simulink model "v2012_PF"  (Simulink 7.6)
(part 1 of 4)
settings: Solver=ode45  StartTime=0.0  StopTime=10.0  RelTol=1e-3
libraries: fm_lib x1
settings Model: Creator=davidusb  LastModifiedBy=davidusb

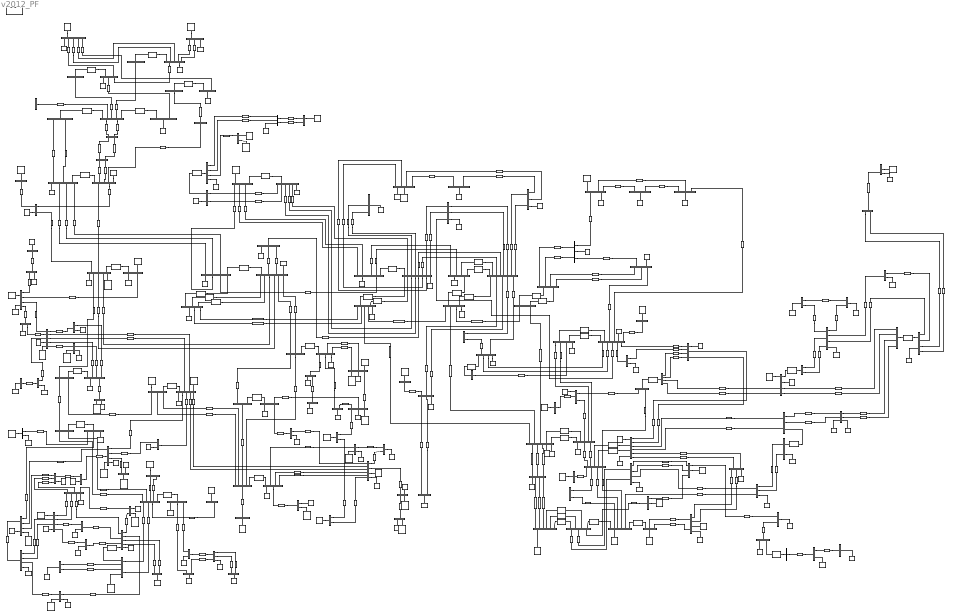
== system v2012_PF ==
  note: Hacia Empresas
      | Mixtas PDVSA
  note: REACTOR
      | 3x300
  note: REACTOR
      | 4x300
  note: COMP
      | ESTATICO
  note: REACTOR
      | 2x50
  note: Guri 400 kV
  note: Macagua I y III
  note: Caruachi
  note: Macagua II
  note: S/E San Geronimo 765kV
  note: S/E Malena 765kV
  note: S/E Guri 765kV
  note: Ciudad
      | Guayana
  note: Guri 230 kV
  note: (AT adicional 150MVA 2012)
  note: 2x100MVAr
      | SHUNT CAP
  note: Puerto La Cruz
  note: Caracas
  note: Maracay
  note: S/E Sur 765kV
  note: REACTOR
      | 2x100
  note: (2da linea 2012)
  note: Valencia
  note: S/E La Horqueta 765kV
  note: S/E La Arenosa 765kV
  note: LIBRE
  note: Elaborado por: Ing. David Hernández Torres, PhD
      |
      | VERSION: 29 de Noviembre de 2012 (Simplificada, niveles de tensión: 765, 400 y 230 kV)
      | (Solo se consideran una pequeña parte de la red oriental y la red de Los Andes en 115kV)
      |
      | Fuentes:
      | Elaborado siguiendo diagrama unifilar actualizado hasta el 2003 (OPSIS) y las actualizaciones
      | del sistema descritas en el Anuario Estadístico del MPPEE hasta el año 2010 y en los
      | informe anuales OPSIS 2005-2008. Finalmente el modelo 2012 se obtiene luego de actualización
      | del modelo 2010 bajo las premisas descritas en los archivos pronostico_demanda_electrica.xls y
      | Datos SEN.xls
      |
      | (Es necesaria la instalación del toolbox PSAT, el esquema se elaboró con Simulink
      | y la version 7.11 R2010b de Matlab, se puede ejecutar el archivo de datos .m desde Octave y la
      | version de PSAT correspondiente)
  note: SISTEMA ELECTRICO NACIONAL
  note: COMP
      | ESTATICO
  note: REACTOR
      | 2x50
  note: REACTOR
      | 1x300
  note: REACTOR
      | 2x25
  note: Cumana
  note: REACTOR
      | 1x50
  note: Isla de Margarita
  note: REACTOR
      | 2x25
  note: Brasil
  note: REACTOR
      | 2x50
  note: TAP=1.1
  note: Termozulia
      | Rafael Urdaneta
  note: CAPACITOR
      | 1x108
  note: REACTOR
      | 1x50
  note: REACTOR
      | 4x50
  note: SERIES
      | CAPACITOR
      | COMP
      | 3x50 OHM
  note: Maracaibo
  note: HACIA COLOMBIA
  note: REACTOR
      | 1x300
  note: REACTOR
      | 4x50
  note: LIBRE
  note: LIBRE
  note: S/E Yaracuy 765kV
  note: Barquisimeto
  note: Merida
  note: San Cristobal
  note: Colombia
  note: REACTOR
      | 2x20
  note: Peninsula de Paraguaná
  note: (2da linea 2012)
  note: (Entrada de 257MW en 2013)
      | Fabricio Ojeda
  note: Equivalente
      | hacia Cabudare
  note: Equivalente
      | hacia Cabimas -
      | El Tablazo
  Acarigua I : PMComponent  Tag=PSATblock  Description=Connection  PhysicalDomain=psatdomain  LeftPortType=p1  RightPortType=p1  LConnTagsString=__newl0|__newl1|__newl2  RConnTagsString=__newr0|__newr1|__newr2  mask(Bus){in=3, out=3, p2q=115, p3_4q=[0.98444    -0.26004], p5q=1, p6q=1}
      mask prompts: in "Number of inputs:"; out "Number of outputs:"; p2q "Voltage Rating [kV]"; p3_4q "Voltage initial guess [p.u.  rad]"; p5q "Area number"; p6q "Region number"
      mask help: Bus block.
      mask init:
      | fm_inout
      settings: AttributesFormatString="|V| =  0.9513 p.u.\\n<V  = -0.0895 rad"
      mask CallbackString: ||||fm_block|
      mask Display: plot([0 1 1 0 0],[0 0 1 1 0])
  Acarigua II 115kV : PMComponent  Tag=PSATblock  Description=Connection  PhysicalDomain=psatdomain  LeftPortType=p1  RightPortType=p1  LConnTagsString=__newl0|__newl1|__newl2  RConnTagsString=__newr0|__newr1|__newr2|__newr3  mask(Bus){in=3, out=4, p2q=115, p3_4q=[0.98444    -0.26004], p5q=1, p6q=1}
      mask prompts: in "Number of inputs:"; out "Number of outputs:"; p2q "Voltage Rating [kV]"; p3_4q "Voltage initial guess [p.u.  rad]"; p5q "Area number"; p6q "Region number"
      mask help: Bus block.
      mask init:
      | fm_inout
      settings: AttributesFormatString="|V| =  0.9304 p.u.\\n<V  = -0.1031 rad"
      mask CallbackString: ||||fm_block|
      mask Display: plot([0 1 1 0 0],[0 0 1 1 0])
  Acarigua II 230kV : PMComponent  Tag=PSATblock  Description=Connection  PhysicalDomain=psatdomain  LeftPortType=p1  RightPortType=p1  LConnTagsString=__newl0|__newl1|__newl2  RConnTagsString=__newr0|__newr1|__newr2  mask(Bus){in=3, out=3, p2q=230, p3_4q=[0.96856    -0.61292], p5q=1, p6q=1}
      mask prompts: in "Number of inputs:"; out "Number of outputs:"; p2q "Voltage Rating [kV]"; p3_4q "Voltage initial guess [p.u.  rad]"; p5q "Area number"; p6q "Region number"
      mask help: Bus block.
      mask init:
      | fm_inout
      settings: AttributesFormatString="|V| =  0.9644 p.u.\\n<V  = -0.0672 rad"
      mask CallbackString: ||||fm_block|
      mask Display: plot([0 1 1 0 0],[0 0 1 1 0])
  Aragua 230kV : PMComponent  Tag=PSATblock  Description=Connection  PhysicalDomain=psatdomain  LeftPortType=p1  RightPortType=p1  LConnTagsString=__newl0|__newl1|__newl2  RConnTagsString=__newr0|__newr1|__newr2  mask(Bus){in=3, out=3, p2q=230, p3_4q=[0.953    -0.54917], p5q=1, p6q=1}
      mask prompts: in "Number of inputs:"; out "Number of outputs:"; p2q "Voltage Rating [kV]"; p3_4q "Voltage initial guess [p.u.  rad]"; p5q "Area number"; p6q "Region number"
      mask help: Bus block.
      mask init:
      | fm_inout
      settings: AttributesFormatString="|V| =  0.9696 p.u.\\n<V  = -0.2355 rad"
      mask CallbackString: ||||fm_block|
      mask Display: plot([0 1 1 0 0],[0 0 1 1 0])
  Araure : PMComponent  Tag=PSATblock  Description=Connection  PhysicalDomain=psatdomain  LeftPortType=p1  RightPortType=p1  LConnTagsString=__newl0|__newl1  RConnTagsString=__newr0  mask(Bus){in=2, out=1, p2q=115, p3_4q=[1.0023    -0.25717], p5q=1, p6q=1}
      mask prompts: in "Number of inputs:"; out "Number of outputs:"; p2q "Voltage Rating [kV]"; p3_4q "Voltage initial guess [p.u.  rad]"; p5q "Area number"; p6q "Region number"
      mask help: Bus block.
      mask init:
      | fm_inout
      settings: AttributesFormatString="|V| =  0.9284 p.u.\\n<V  = -0.0990 rad"
      mask CallbackString: ||||fm_block|
      mask Display: plot([0 1 1 0 0],[0 0 1 1 0])
  Auto1 : PMComponent  Tag=PSATblock  Description=Power Flow  PhysicalDomain=psatdomain  LeftPortType=p1  RightPortType=p1  LConnTagsString=__newl0  RConnTagsString=__newr0  mask(Line){p3_4_5q=[1500  765 60], p7q=1.9124, p8q=0.003, p9q=0.148, p13_14_15q=[0.0  0.0  0.0], p16q=on}
      mask prompts: p3_4_5q "Power, Voltage and Frequency Ratings [MVA, kV, Hz]"; p7q "Primary and secondary voltage ratio [kV/kV]"; p8q "Resistance [p.u.]"; p9q "Reactance [p.u.]"; p13_14_15q "Imax, Pmax and Smax [p.u., p.u., p.u.]"; p16q "Connected"
      mask help: This block defines an auto-transformer.
      mask init:
      | [x,y] = fm_draw('circle');
      | [xq,yq] = fm_draw('quarter');
      mask CallbackString: |||||fm_block
      mask Display: plot(x,y,1.75*xq,yq,[-1 -1.3],[0 0],[1.75 2.05],[0 0])
  Auto10 : PMComponent  Tag=PSATblock  Description=Power Flow  PhysicalDomain=psatdomain  LeftPortType=p1  RightPortType=p1  LConnTagsString=__newl0  RConnTagsString=__newr0  mask(Line){p3_4_5q=[200  230 60], p7q=2, p8q=0.01, p9q=0.16, p13_14_15q=[0.0  0.0  0.0], p16q=on}
      mask prompts: p3_4_5q "Power, Voltage and Frequency Ratings [MVA, kV, Hz]"; p7q "Primary and secondary voltage ratio [kV/kV]"; p8q "Resistance [p.u.]"; p9q "Reactance [p.u.]"; p13_14_15q "Imax, Pmax and Smax [p.u., p.u., p.u.]"; p16q "Connected"
      mask help: This block defines an auto-transformer.
      mask init:
      | [x,y] = fm_draw('circle');
      | [xq,yq] = fm_draw('quarter');
      mask CallbackString: |||||fm_block
      mask Display: plot(x,y,1.75*xq,yq,[-1 -1.3],[0 0],[1.75 2.05],[0 0])
  Auto11 : PMComponent  Tag=PSATblock  Description=Power Flow  PhysicalDomain=psatdomain  LeftPortType=p1  RightPortType=p1  LConnTagsString=__newl0  RConnTagsString=__newr0  mask(Line){p3_4_5q=[900  400 60], p7q=1.7391, p8q=0.0024, p9q=0.10, p13_14_15q=[0.0  0.0  0.0], p16q=on}
      mask prompts: p3_4_5q "Power, Voltage and Frequency Ratings [MVA, kV, Hz]"; p7q "Primary and secondary voltage ratio [kV/kV]"; p8q "Resistance [p.u.]"; p9q "Reactance [p.u.]"; p13_14_15q "Imax, Pmax and Smax [p.u., p.u., p.u.]"; p16q "Connected"
      mask help: This block defines an auto-transformer.
      mask init:
      | [x,y] = fm_draw('circle');
      | [xq,yq] = fm_draw('quarter');
      mask CallbackString: |||||fm_block
      mask Display: plot(x,y,1.75*xq,yq,[-1 -1.3],[0 0],[1.75 2.05],[0 0])
  Auto12 : PMComponent  Tag=PSATblock  Description=Power Flow  PhysicalDomain=psatdomain  LeftPortType=p1  RightPortType=p1  LConnTagsString=__newl0  RConnTagsString=__newr0  mask(Line){p3_4_5q=[100  230 60], p7q=2, p8q=0.01, p9q=0.16, p13_14_15q=[0.0  0.0  0.0], p16q=on}
      mask prompts: p3_4_5q "Power, Voltage and Frequency Ratings [MVA, kV, Hz]"; p7q "Primary and secondary voltage ratio [kV/kV]"; p8q "Resistance [p.u.]"; p9q "Reactance [p.u.]"; p13_14_15q "Imax, Pmax and Smax [p.u., p.u., p.u.]"; p16q "Connected"
      mask help: This block defines an auto-transformer.
      mask init:
      | [x,y] = fm_draw('circle');
      | [xq,yq] = fm_draw('quarter');
      mask CallbackString: |||||fm_block
      mask Display: plot(x,y,1.75*xq,yq,[-1 -1.3],[0 0],[1.75 2.05],[0 0])
  Auto13 : PMComponent  Tag=PSATblock  Description=Power Flow  PhysicalDomain=psatdomain  LeftPortType=p1  RightPortType=p1  LConnTagsString=__newl0  RConnTagsString=__newr0  mask(Line){p3_4_5q=[200  230 60], p7q=2, p8q=0.01, p9q=0.16, p13_14_15q=[0.0  0.0  0.0], p16q=on}
      mask prompts: p3_4_5q "Power, Voltage and Frequency Ratings [MVA, kV, Hz]"; p7q "Primary and secondary voltage ratio [kV/kV]"; p8q "Resistance [p.u.]"; p9q "Reactance [p.u.]"; p13_14_15q "Imax, Pmax and Smax [p.u., p.u., p.u.]"; p16q "Connected"
      mask help: This block defines an auto-transformer.
      mask init:
      | [x,y] = fm_draw('circle');
      | [xq,yq] = fm_draw('quarter');
      mask CallbackString: |||||fm_block
      mask Display: plot(x,y,1.75*xq,yq,[-1 -1.3],[0 0],[1.75 2.05],[0 0])
  Auto14 : PMComponent  Tag=PSATblock  Description=Power Flow  PhysicalDomain=psatdomain  LeftPortType=p1  RightPortType=p1  LConnTagsString=__newl0  RConnTagsString=__newr0  mask(Line){p3_4_5q=[400  230 60], p7q=2, p8q=0.01, p9q=0.16, p13_14_15q=[0.0  0.0  0.0], p16q=on}
      mask prompts: p3_4_5q "Power, Voltage and Frequency Ratings [MVA, kV, Hz]"; p7q "Primary and secondary voltage ratio [kV/kV]"; p8q "Resistance [p.u.]"; p9q "Reactance [p.u.]"; p13_14_15q "Imax, Pmax and Smax [p.u., p.u., p.u.]"; p16q "Connected"
      mask help: This block defines an auto-transformer.
      mask init:
      | [x,y] = fm_draw('circle');
      | [xq,yq] = fm_draw('quarter');
      mask CallbackString: |||||fm_block
      mask Display: plot(x,y,1.75*xq,yq,[-1 -1.3],[0 0],[1.75 2.05],[0 0])
  Auto15 : PMComponent  Tag=PSATblock  Description=Power Flow  PhysicalDomain=psatdomain  LeftPortType=p1  RightPortType=p1  LConnTagsString=__newl0  RConnTagsString=__newr0  mask(Line){p3_4_5q=[1500  765 60], p7q=1.9124, p8q=0.003, p9q=0.148, p13_14_15q=[0.0  0.0  0.0], p16q=on}
      mask prompts: p3_4_5q "Power, Voltage and Frequency Ratings [MVA, kV, Hz]"; p7q "Primary and secondary voltage ratio [kV/kV]"; p8q "Resistance [p.u.]"; p9q "Reactance [p.u.]"; p13_14_15q "Imax, Pmax and Smax [p.u., p.u., p.u.]"; p16q "Connected"
      mask help: This block defines an auto-transformer.
      mask init:
      | [x,y] = fm_draw('circle');
      | [xq,yq] = fm_draw('quarter');
      mask CallbackString: |||||fm_block
      mask Display: plot(x,y,1.75*xq,yq,[-1 -1.3],[0 0],[1.75 2.05],[0 0])
  Auto16 : PMComponent  Tag=PSATblock  Description=Power Flow  PhysicalDomain=psatdomain  LeftPortType=p1  RightPortType=p1  LConnTagsString=__newl0  RConnTagsString=__newr0  mask(Line){p3_4_5q=[1000  400 60], p7q=1, p8q=0.001, p9q=0.0513, p13_14_15q=[0.0  0.0  0.0], p16q=on}
      mask prompts: p3_4_5q "Power, Voltage and Frequency Ratings [MVA, kV, Hz]"; p7q "Primary and secondary voltage ratio [kV/kV]"; p8q "Resistance [p.u.]"; p9q "Reactance [p.u.]"; p13_14_15q "Imax, Pmax and Smax [p.u., p.u., p.u.]"; p16q "Connected"
      mask help: This block defines an auto-transformer.
      mask init:
      | [x,y] = fm_draw('circle');
      | [xq,yq] = fm_draw('quarter');
      mask CallbackString: |||||fm_block
      mask Display: plot(x,y,1.75*xq,yq,[-1 -1.3],[0 0],[1.75 2.05],[0 0])
  Auto17 : PMComponent  Tag=PSATblock  Description=Power Flow  PhysicalDomain=psatdomain  LeftPortType=p1  RightPortType=p1  LConnTagsString=__newl0  RConnTagsString=__newr0  mask(Line){p3_4_5q=[450  400 60], p7q=1.7391, p8q=0.002, p9q=0.10, p13_14_15q=[0.0  0.0  0.0], p16q=on}
      mask prompts: p3_4_5q "Power, Voltage and Frequency Ratings [MVA, kV, Hz]"; p7q "Primary and secondary voltage ratio [kV/kV]"; p8q "Resistance [p.u.]"; p9q "Reactance [p.u.]"; p13_14_15q "Imax, Pmax and Smax [p.u., p.u., p.u.]"; p16q "Connected"
      mask help: This block defines an auto-transformer.
      mask init:
      | [x,y] = fm_draw('circle');
      | [xq,yq] = fm_draw('quarter');
      mask CallbackString: |||||fm_block
      mask Display: plot(x,y,1.75*xq,yq,[-1 -1.3],[0 0],[1.75 2.05],[0 0])
  Auto18 : PMComponent  Tag=PSATblock  Description=Power Flow  PhysicalDomain=psatdomain  LeftPortType=p1  RightPortType=p1  LConnTagsString=__newl0  RConnTagsString=__newr0  mask(Line){p3_4_5q=[450  400 60], p7q=1.7391, p8q=0.0011, p9q=0.0546, p13_14_15q=[0.0  0.0  0.0], p16q=on}
      mask prompts: p3_4_5q "Power, Voltage and Frequency Ratings [MVA, kV, Hz]"; p7q "Primary and secondary voltage ratio [kV/kV]"; p8q "Resistance [p.u.]"; p9q "Reactance [p.u.]"; p13_14_15q "Imax, Pmax and Smax [p.u., p.u., p.u.]"; p16q "Connected"
      mask help: This block defines an auto-transformer.
      mask init:
      | [x,y] = fm_draw('circle');
      | [xq,yq] = fm_draw('quarter');
      mask CallbackString: |||||fm_block
      mask Display: plot(x,y,1.75*xq,yq,[-1 -1.3],[0 0],[1.75 2.05],[0 0])
  Auto19 : PMComponent  Tag=PSATblock  Description=Power Flow  PhysicalDomain=psatdomain  LeftPortType=p1  RightPortType=p1  LConnTagsString=__newl0  RConnTagsString=__newr0  mask(Line){p3_4_5q=[1000  765 60], p7q=3.3256, p8q=0.003, p9q=0.15, p13_14_15q=[0.0  0.0  0.0], p16q=on}
      mask prompts: p3_4_5q "Power, Voltage and Frequency Ratings [MVA, kV, Hz]"; p7q "Primary and secondary voltage ratio [kV/kV]"; p8q "Resistance [p.u.]"; p9q "Reactance [p.u.]"; p13_14_15q "Imax, Pmax and Smax [p.u., p.u., p.u.]"; p16q "Connected"
      mask help: This block defines an auto-transformer.
      mask init:
      | [x,y] = fm_draw('circle');
      | [xq,yq] = fm_draw('quarter');
      mask CallbackString: |||||fm_block
      mask Display: plot(x,y,1.75*xq,yq,[-1 -1.3],[0 0],[1.75 2.05],[0 0])
  Auto2 : PMComponent  Tag=PSATblock  Description=Power Flow  PhysicalDomain=psatdomain  LeftPortType=p1  RightPortType=p1  LConnTagsString=__newl0  RConnTagsString=__newr0  mask(Line){p3_4_5q=[1500  765 60], p7q=1.9124, p8q=0.003, p9q=0.148, p13_14_15q=[0.0  0.0  0.0], p16q=on}
      mask prompts: p3_4_5q "Power, Voltage and Frequency Ratings [MVA, kV, Hz]"; p7q "Primary and secondary voltage ratio [kV/kV]"; p8q "Resistance [p.u.]"; p9q "Reactance [p.u.]"; p13_14_15q "Imax, Pmax and Smax [p.u., p.u., p.u.]"; p16q "Connected"
      mask help: This block defines an auto-transformer.
      mask init:
      | [x,y] = fm_draw('circle');
      | [xq,yq] = fm_draw('quarter');
      mask CallbackString: |||||fm_block
      mask Display: plot(x,y,1.75*xq,yq,[-1 -1.3],[0 0],[1.75 2.05],[0 0])
  Auto20 : PMComponent  Tag=PSATblock  Description=Power Flow  PhysicalDomain=psatdomain  LeftPortType=p1  RightPortType=p1  LConnTagsString=__newl0  RConnTagsString=__newr0  mask(Line){p3_4_5q=[450  400 60], p7q=1.7391, p8q=0.0011, p9q=0.0546, p13_14_15q=[0.0  0.0  0.0], p16q=on}
      mask prompts: p3_4_5q "Power, Voltage and Frequency Ratings [MVA, kV, Hz]"; p7q "Primary and secondary voltage ratio [kV/kV]"; p8q "Resistance [p.u.]"; p9q "Reactance [p.u.]"; p13_14_15q "Imax, Pmax and Smax [p.u., p.u., p.u.]"; p16q "Connected"
      mask help: This block defines an auto-transformer.
      mask init:
      | [x,y] = fm_draw('circle');
      | [xq,yq] = fm_draw('quarter');
      mask CallbackString: |||||fm_block
      mask Display: plot(x,y,1.75*xq,yq,[-1 -1.3],[0 0],[1.75 2.05],[0 0])
  Auto21 : PMComponent  Tag=PSATblock  Description=Power Flow  PhysicalDomain=psatdomain  LeftPortType=p1  RightPortType=p1  LConnTagsString=__newl0  RConnTagsString=__newr0  mask(Line){p3_4_5q=[450 400 60], p7q=1.7391, p8q=0.003, p9q=0.15, p13_14_15q=[0.0  0.0  0.0], p16q=on}
      mask prompts: p3_4_5q "Power, Voltage and Frequency Ratings [MVA, kV, Hz]"; p7q "Primary and secondary voltage ratio [kV/kV]"; p8q "Resistance [p.u.]"; p9q "Reactance [p.u.]"; p13_14_15q "Imax, Pmax and Smax [p.u., p.u., p.u.]"; p16q "Connected"
      mask help: This block defines an auto-transformer.
      mask init:
      | [x,y] = fm_draw('circle');
      | [xq,yq] = fm_draw('quarter');
      mask CallbackString: |||||fm_block
      mask Display: plot(x,y,1.75*xq,yq,[-1 -1.3],[0 0],[1.75 2.05],[0 0])
  Auto22 : PMComponent  Tag=PSATblock  Description=Power Flow  PhysicalDomain=psatdomain  LeftPortType=p1  RightPortType=p1  LConnTagsString=__newl0  RConnTagsString=__newr0  mask(Line){p3_4_5q=[1000  765 60], p7q=3.3256, p8q=0.003, p9q=0.15, p13_14_15q=[0.0  0.0  0.0], p16q=on}
      mask prompts: p3_4_5q "Power, Voltage and Frequency Ratings [MVA, kV, Hz]"; p7q "Primary and secondary voltage ratio [kV/kV]"; p8q "Resistance [p.u.]"; p9q "Reactance [p.u.]"; p13_14_15q "Imax, Pmax and Smax [p.u., p.u., p.u.]"; p16q "Connected"
      mask help: This block defines an auto-transformer.
      mask init:
      | [x,y] = fm_draw('circle');
      | [xq,yq] = fm_draw('quarter');
      mask CallbackString: |||||fm_block
      mask Display: plot(x,y,1.75*xq,yq,[-1 -1.3],[0 0],[1.75 2.05],[0 0])
  Auto23 : PMComponent  Tag=PSATblock  Description=Power Flow  PhysicalDomain=psatdomain  LeftPortType=p1  RightPortType=p1  LConnTagsString=__newl0  RConnTagsString=__newr0  mask(Line){p3_4_5q=[1500  765 60], p7q=1.9124, p8q=0.003, p9q=0.148, p13_14_15q=[0.0  0.0  0.0], p16q=on}
      mask prompts: p3_4_5q "Power, Voltage and Frequency Ratings [MVA, kV, Hz]"; p7q "Primary and secondary voltage ratio [kV/kV]"; p8q "Resistance [p.u.]"; p9q "Reactance [p.u.]"; p13_14_15q "Imax, Pmax and Smax [p.u., p.u., p.u.]"; p16q "Connected"
      mask help: This block defines an auto-transformer.
      mask init:
      | [x,y] = fm_draw('circle');
      | [xq,yq] = fm_draw('quarter');
      mask CallbackString: |||||fm_block
      mask Display: plot(x,y,1.75*xq,yq,[-1 -1.3],[0 0],[1.75 2.05],[0 0])
  Auto24 : PMComponent  Tag=PSATblock  Description=Power Flow  PhysicalDomain=psatdomain  LeftPortType=p1  RightPortType=p1  LConnTagsString=__newl0  RConnTagsString=__newr0  mask(Line){p3_4_5q=[1000 765 60], p7q=3.3256, p8q=0.003, p9q=0.15, p13_14_15q=[0.0  0.0  0.0], p16q=on}
      mask prompts: p3_4_5q "Power, Voltage and Frequency Ratings [MVA, kV, Hz]"; p7q "Primary and secondary voltage ratio [kV/kV]"; p8q "Resistance [p.u.]"; p9q "Reactance [p.u.]"; p13_14_15q "Imax, Pmax and Smax [p.u., p.u., p.u.]"; p16q "Connected"
      mask help: This block defines an auto-transformer.
      mask init:
      | [x,y] = fm_draw('circle');
      | [xq,yq] = fm_draw('quarter');
      mask CallbackString: |||||fm_block
      mask Display: plot(x,y,1.75*xq,yq,[-1 -1.3],[0 0],[1.75 2.05],[0 0])
  Auto25 : PMComponent  Tag=PSATblock  Description=Power Flow  PhysicalDomain=psatdomain  LeftPortType=p1  RightPortType=p1  LConnTagsString=__newl0  RConnTagsString=__newr0  mask(Line){p3_4_5q=[450 400 60], p7q=1.7391, p8q=0.003, p9q=0.15, p13_14_15q=[0.0  0.0  0.0], p16q=on}
      mask prompts: p3_4_5q "Power, Voltage and Frequency Ratings [MVA, kV, Hz]"; p7q "Primary and secondary voltage ratio [kV/kV]"; p8q "Resistance [p.u.]"; p9q "Reactance [p.u.]"; p13_14_15q "Imax, Pmax and Smax [p.u., p.u., p.u.]"; p16q "Connected"
      mask help: This block defines an auto-transformer.
      mask init:
      | [x,y] = fm_draw('circle');
      | [xq,yq] = fm_draw('quarter');
      mask CallbackString: |||||fm_block
      mask Display: plot(x,y,1.75*xq,yq,[-1 -1.3],[0 0],[1.75 2.05],[0 0])
  Auto26 : PMComponent  Tag=PSATblock  Description=Power Flow  PhysicalDomain=psatdomain  LeftPortType=p1  RightPortType=p1  LConnTagsString=__newl0  RConnTagsString=__newr0  mask(Line){p3_4_5q=[1000 765 60], p7q=3.3256, p8q=0.003, p9q=0.15, p13_14_15q=[0.0  0.0  0.0], p16q=on}
      mask prompts: p3_4_5q "Power, Voltage and Frequency Ratings [MVA, kV, Hz]"; p7q "Primary and secondary voltage ratio [kV/kV]"; p8q "Resistance [p.u.]"; p9q "Reactance [p.u.]"; p13_14_15q "Imax, Pmax and Smax [p.u., p.u., p.u.]"; p16q "Connected"
      mask help: This block defines an auto-transformer.
      mask init:
      | [x,y] = fm_draw('circle');
      | [xq,yq] = fm_draw('quarter');
      mask CallbackString: |||||fm_block
      mask Display: plot(x,y,1.75*xq,yq,[-1 -1.3],[0 0],[1.75 2.05],[0 0])
  Auto27 : PMComponent  Tag=PSATblock  Description=Power Flow  PhysicalDomain=psatdomain  LeftPortType=p1  RightPortType=p1  LConnTagsString=__newl0  RConnTagsString=__newr0  mask(Line){p3_4_5q=[333 230 60], p7q=1.6666, p8q=0.01, p9q=0.16, p13_14_15q=[0.0  0.0  0.0], p16q=on}
      mask prompts: p3_4_5q "Power, Voltage and Frequency Ratings [MVA, kV, Hz]"; p7q "Primary and secondary voltage ratio [kV/kV]"; p8q "Resistance [p.u.]"; p9q "Reactance [p.u.]"; p13_14_15q "Imax, Pmax and Smax [p.u., p.u., p.u.]"; p16q "Connected"
      mask help: This block defines an auto-transformer.
      mask init:
      | [x,y] = fm_draw('circle');
      | [xq,yq] = fm_draw('quarter');
      mask CallbackString: |||||fm_block
      mask Display: plot(x,y,1.75*xq,yq,[-1 -1.3],[0 0],[1.75 2.05],[0 0])
  Auto28 : PMComponent  Tag=PSATblock  Description=Power Flow  PhysicalDomain=psatdomain  LeftPortType=p1  RightPortType=p1  LConnTagsString=__newl0  RConnTagsString=__newr0  mask(Line){p3_4_5q=[1000 765 60], p7q=3.3256, p8q=0.003, p9q=0.15, p13_14_15q=[0.0  0.0  0.0], p16q=on}
      mask prompts: p3_4_5q "Power, Voltage and Frequency Ratings [MVA, kV, Hz]"; p7q "Primary and secondary voltage ratio [kV/kV]"; p8q "Resistance [p.u.]"; p9q "Reactance [p.u.]"; p13_14_15q "Imax, Pmax and Smax [p.u., p.u., p.u.]"; p16q "Connected"
      mask help: This block defines an auto-transformer.
      mask init:
      | [x,y] = fm_draw('circle');
      | [xq,yq] = fm_draw('quarter');
      mask CallbackString: |||||fm_block
      mask Display: plot(x,y,1.75*xq,yq,[-1 -1.3],[0 0],[1.75 2.05],[0 0])
  Auto29 : PMComponent  Tag=PSATblock  Description=Power Flow  PhysicalDomain=psatdomain  LeftPortType=p1  RightPortType=p1  LConnTagsString=__newl0  RConnTagsString=__newr0  mask(Line){p3_4_5q=[900 400 60], p7q=1.7391, p8q=0.001, p9q=0.0513, p13_14_15q=[0.0  0.0  0.0], p16q=on}
      mask prompts: p3_4_5q "Power, Voltage and Frequency Ratings [MVA, kV, Hz]"; p7q "Primary and secondary voltage ratio [kV/kV]"; p8q "Resistance [p.u.]"; p9q "Reactance [p.u.]"; p13_14_15q "Imax, Pmax and Smax [p.u., p.u., p.u.]"; p16q "Connected"
      mask help: This block defines an auto-transformer.
      mask init:
      | [x,y] = fm_draw('circle');
      | [xq,yq] = fm_draw('quarter');
      mask CallbackString: |||||fm_block
      mask Display: plot(x,y,1.75*xq,yq,[-1 -1.3],[0 0],[1.75 2.05],[0 0])
  Auto3 : PMComponent  Tag=PSATblock  Description=Power Flow  PhysicalDomain=psatdomain  LeftPortType=p1  RightPortType=p1  LConnTagsString=__newl0  RConnTagsString=__newr0  mask(Line){p3_4_5q=[450  400 60], p7q=1.7391, p8q=0.001, p9q=0.0513, p13_14_15q=[0.0  0.0  0.0], p16q=on}
      mask prompts: p3_4_5q "Power, Voltage and Frequency Ratings [MVA, kV, Hz]"; p7q "Primary and secondary voltage ratio [kV/kV]"; p8q "Resistance [p.u.]"; p9q "Reactance [p.u.]"; p13_14_15q "Imax, Pmax and Smax [p.u., p.u., p.u.]"; p16q "Connected"
      mask help: This block defines an auto-transformer.
      mask init:
      | [x,y] = fm_draw('circle');
      | [xq,yq] = fm_draw('quarter');
      mask CallbackString: |||||fm_block
      mask Display: plot(x,y,1.75*xq,yq,[-1 -1.3],[0 0],[1.75 2.05],[0 0])
  Auto30 : PMComponent  Tag=PSATblock  Description=Power Flow  PhysicalDomain=psatdomain  LeftPortType=p1  RightPortType=p1  LConnTagsString=__newl0  RConnTagsString=__newr0  mask(Line){p3_4_5q=[333 230 60], p7q=1.6666, p8q=0.01, p9q=0.16, p13_14_15q=[0.0  0.0  0.0], p16q=on}
      mask prompts: p3_4_5q "Power, Voltage and Frequency Ratings [MVA, kV, Hz]"; p7q "Primary and secondary voltage ratio [kV/kV]"; p8q "Resistance [p.u.]"; p9q "Reactance [p.u.]"; p13_14_15q "Imax, Pmax and Smax [p.u., p.u., p.u.]"; p16q "Connected"
      mask help: This block defines an auto-transformer.
      mask init:
      | [x,y] = fm_draw('circle');
      | [xq,yq] = fm_draw('quarter');
      mask CallbackString: |||||fm_block
      mask Display: plot(x,y,1.75*xq,yq,[-1 -1.3],[0 0],[1.75 2.05],[0 0])
  Auto31 : PMComponent  Tag=PSATblock  Description=Power Flow  PhysicalDomain=psatdomain  LeftPortType=p1  RightPortType=p1  LConnTagsString=__newl0  RConnTagsString=__newr0  mask(Line){p3_4_5q=[333 230 60], p7q=1.6666, p8q=0.01, p9q=0.16, p13_14_15q=[0.0  0.0  0.0], p16q=on}
      mask prompts: p3_4_5q "Power, Voltage and Frequency Ratings [MVA, kV, Hz]"; p7q "Primary and secondary voltage ratio [kV/kV]"; p8q "Resistance [p.u.]"; p9q "Reactance [p.u.]"; p13_14_15q "Imax, Pmax and Smax [p.u., p.u., p.u.]"; p16q "Connected"
      mask help: This block defines an auto-transformer.
      mask init:
      | [x,y] = fm_draw('circle');
      | [xq,yq] = fm_draw('quarter');
      mask CallbackString: |||||fm_block
      mask Display: plot(x,y,1.75*xq,yq,[-1 -1.3],[0 0],[1.75 2.05],[0 0])
  Auto37 : PMComponent  Tag=PSATblock  Description=Power Flow  PhysicalDomain=psatdomain  LeftPortType=p1  RightPortType=p1  LConnTagsString=__newl0  RConnTagsString=__newr0  mask(Line){p3_4_5q=[450 400 60], p7q=1.7391, p8q=0.002, p9q=0.10, p13_14_15q=[0.0  0.0  0.0], p16q=on}
      mask prompts: p3_4_5q "Power, Voltage and Frequency Ratings [MVA, kV, Hz]"; p7q "Primary and secondary voltage ratio [kV/kV]"; p8q "Resistance [p.u.]"; p9q "Reactance [p.u.]"; p13_14_15q "Imax, Pmax and Smax [p.u., p.u., p.u.]"; p16q "Connected"
      mask help: This block defines an auto-transformer.
      mask init:
      | [x,y] = fm_draw('circle');
      | [xq,yq] = fm_draw('quarter');
      mask CallbackString: |||||fm_block
      mask Display: plot(x,y,1.75*xq,yq,[-1 -1.3],[0 0],[1.75 2.05],[0 0])
  Auto38 : PMComponent  Tag=PSATblock  Description=Power Flow  PhysicalDomain=psatdomain  LeftPortType=p1  RightPortType=p1  LConnTagsString=__newl0  RConnTagsString=__newr0  mask(Line){p3_4_5q=[1500  765 60], p7q=1.9124, p8q=0.003, p9q=0.148, p13_14_15q=[0.0  0.0  0.0], p16q=on}
      mask prompts: p3_4_5q "Power, Voltage and Frequency Ratings [MVA, kV, Hz]"; p7q "Primary and secondary voltage ratio [kV/kV]"; p8q "Resistance [p.u.]"; p9q "Reactance [p.u.]"; p13_14_15q "Imax, Pmax and Smax [p.u., p.u., p.u.]"; p16q "Connected"
      mask help: This block defines an auto-transformer.
      mask init:
      | [x,y] = fm_draw('circle');
      | [xq,yq] = fm_draw('quarter');
      mask CallbackString: |||||fm_block
      mask Display: plot(x,y,1.75*xq,yq,[-1 -1.3],[0 0],[1.75 2.05],[0 0])
  Auto39 : PMComponent  Tag=PSATblock  Description=Power Flow  PhysicalDomain=psatdomain  LeftPortType=p1  RightPortType=p1  LConnTagsString=__newl0  RConnTagsString=__newr0  mask(Line){p3_4_5q=[1000 765 60], p7q=3.3256, p8q=0.01, p9q=0.21, p13_14_15q=[0.0  0.0  0.0], p16q=on}
      mask prompts: p3_4_5q "Power, Voltage and Frequency Ratings [MVA, kV, Hz]"; p7q "Primary and secondary voltage ratio [kV/kV]"; p8q "Resistance [p.u.]"; p9q "Reactance [p.u.]"; p13_14_15q "Imax, Pmax and Smax [p.u., p.u., p.u.]"; p16q "Connected"
      mask help: This block defines an auto-transformer.
      mask init:
      | [x,y] = fm_draw('circle');
      | [xq,yq] = fm_draw('quarter');
      mask CallbackString: |||||fm_block
      mask Display: plot(x,y,1.75*xq,yq,[-1 -1.3],[0 0],[1.75 2.05],[0 0])
  Auto4 : PMComponent  Tag=PSATblock  Description=Power Flow  PhysicalDomain=psatdomain  LeftPortType=p1  RightPortType=p1  LConnTagsString=__newl0  RConnTagsString=__newr0  mask(Line){p3_4_5q=[1500  765 60], p7q=1.9124, p8q=0.003, p9q=0.149, p13_14_15q=[0.0  0.0  0.0], p16q=on}
      mask prompts: p3_4_5q "Power, Voltage and Frequency Ratings [MVA, kV, Hz]"; p7q "Primary and secondary voltage ratio [kV/kV]"; p8q "Resistance [p.u.]"; p9q "Reactance [p.u.]"; p13_14_15q "Imax, Pmax and Smax [p.u., p.u., p.u.]"; p16q "Connected"
      mask help: This block defines an auto-transformer.
      mask init:
      | [x,y] = fm_draw('circle');
      | [xq,yq] = fm_draw('quarter');
      mask CallbackString: |||||fm_block
      mask Display: plot(x,y,1.75*xq,yq,[-1 -1.3],[0 0],[1.75 2.05],[0 0])
  Auto40 : PMComponent  Tag=PSATblock  Description=Power Flow  PhysicalDomain=psatdomain  LeftPortType=p1  RightPortType=p1  LConnTagsString=__newl0  RConnTagsString=__newr0  mask(Line){p3_4_5q=[900 400 60], p7q=1.7391, p8q=0.001, p9q=0.0495, p13_14_15q=[0.0  0.0  0.0], p16q=on}
      mask prompts: p3_4_5q "Power, Voltage and Frequency Ratings [MVA, kV, Hz]"; p7q "Primary and secondary voltage ratio [kV/kV]"; p8q "Resistance [p.u.]"; p9q "Reactance [p.u.]"; p13_14_15q "Imax, Pmax and Smax [p.u., p.u., p.u.]"; p16q "Connected"
      mask help: This block defines an auto-transformer.
      mask init:
      | [x,y] = fm_draw('circle');
      | [xq,yq] = fm_draw('quarter');
      mask CallbackString: |||||fm_block
      mask Display: plot(x,y,1.75*xq,yq,[-1 -1.3],[0 0],[1.75 2.05],[0 0])
  Auto43 : PMComponent  Tag=PSATblock  Description=Power Flow  PhysicalDomain=psatdomain  LeftPortType=p1  RightPortType=p1  LConnTagsString=__newl0  RConnTagsString=__newr0  mask(Line){p3_4_5q=[100  230 60], p7q=2, p8q=0.01, p9q=0.16, p13_14_15q=[0.0  0.0  0.0], p16q=on}
      mask prompts: p3_4_5q "Power, Voltage and Frequency Ratings [MVA, kV, Hz]"; p7q "Primary and secondary voltage ratio [kV/kV]"; p8q "Resistance [p.u.]"; p9q "Reactance [p.u.]"; p13_14_15q "Imax, Pmax and Smax [p.u., p.u., p.u.]"; p16q "Connected"
      mask help: This block defines an auto-transformer.
      mask init:
      | [x,y] = fm_draw('circle');
      | [xq,yq] = fm_draw('quarter');
      mask CallbackString: |||||fm_block
      mask Display: plot(x,y,1.75*xq,yq,[-1 -1.3],[0 0],[1.75 2.05],[0 0])
  Auto44 : PMComponent  Tag=PSATblock  Description=Power Flow  PhysicalDomain=psatdomain  LeftPortType=p1  RightPortType=p1  LConnTagsString=__newl0  RConnTagsString=__newr0  mask(Line){p3_4_5q=[100  230 60], p7q=2, p8q=0.01, p9q=0.16, p13_14_15q=[0.0  0.0  0.0], p16q=on}
      mask prompts: p3_4_5q "Power, Voltage and Frequency Ratings [MVA, kV, Hz]"; p7q "Primary and secondary voltage ratio [kV/kV]"; p8q "Resistance [p.u.]"; p9q "Reactance [p.u.]"; p13_14_15q "Imax, Pmax and Smax [p.u., p.u., p.u.]"; p16q "Connected"
      mask help: This block defines an auto-transformer.
      mask init:
      | [x,y] = fm_draw('circle');
      | [xq,yq] = fm_draw('quarter');
      mask CallbackString: |||||fm_block
      mask Display: plot(x,y,1.75*xq,yq,[-1 -1.3],[0 0],[1.75 2.05],[0 0])
  Auto45 : PMComponent  Tag=PSATblock  Description=Power Flow  PhysicalDomain=psatdomain  LeftPortType=p1  RightPortType=p1  LConnTagsString=__newl0  RConnTagsString=__newr0  mask(Line){p3_4_5q=[200  230 60], p7q=2, p8q=0.01, p9q=0.16, p13_14_15q=[0.0  0.0  0.0], p16q=on}
      mask prompts: p3_4_5q "Power, Voltage and Frequency Ratings [MVA, kV, Hz]"; p7q "Primary and secondary voltage ratio [kV/kV]"; p8q "Resistance [p.u.]"; p9q "Reactance [p.u.]"; p13_14_15q "Imax, Pmax and Smax [p.u., p.u., p.u.]"; p16q "Connected"
      mask help: This block defines an auto-transformer.
      mask init:
      | [x,y] = fm_draw('circle');
      | [xq,yq] = fm_draw('quarter');
      mask CallbackString: |||||fm_block
      mask Display: plot(x,y,1.75*xq,yq,[-1 -1.3],[0 0],[1.75 2.05],[0 0])
  Auto46 : PMComponent  Tag=PSATblock  Description=Power Flow  PhysicalDomain=psatdomain  LeftPortType=p1  RightPortType=p1  LConnTagsString=__newl0  RConnTagsString=__newr0  mask(Line){p3_4_5q=[150  230 60], p7q=2, p8q=0.01, p9q=0.16, p13_14_15q=[0.0  0.0  0.0], p16q=on}
      mask prompts: p3_4_5q "Power, Voltage and Frequency Ratings [MVA, kV, Hz]"; p7q "Primary and secondary voltage ratio [kV/kV]"; p8q "Resistance [p.u.]"; p9q "Reactance [p.u.]"; p13_14_15q "Imax, Pmax and Smax [p.u., p.u., p.u.]"; p16q "Connected"
      mask help: This block defines an auto-transformer.
      mask init:
      | [x,y] = fm_draw('circle');
      | [xq,yq] = fm_draw('quarter');
      mask CallbackString: |||||fm_block
      mask Display: plot(x,y,1.75*xq,yq,[-1 -1.3],[0 0],[1.75 2.05],[0 0])
  Auto47 : PMComponent  Tag=PSATblock  Description=Power Flow  PhysicalDomain=psatdomain  LeftPortType=p1  RightPortType=p1  LConnTagsString=__newl0  RConnTagsString=__newr0  mask(Line){p3_4_5q=[250  230 60], p7q=2, p8q=0.01, p9q=0.16, p13_14_15q=[0.0  0.0  0.0], p16q=on}
      mask prompts: p3_4_5q "Power, Voltage and Frequency Ratings [MVA, kV, Hz]"; p7q "Primary and secondary voltage ratio [kV/kV]"; p8q "Resistance [p.u.]"; p9q "Reactance [p.u.]"; p13_14_15q "Imax, Pmax and Smax [p.u., p.u., p.u.]"; p16q "Connected"
      mask help: This block defines an auto-transformer.
      mask init:
      | [x,y] = fm_draw('circle');
      | [xq,yq] = fm_draw('quarter');
      mask CallbackString: |||||fm_block
      mask Display: plot(x,y,1.75*xq,yq,[-1 -1.3],[0 0],[1.75 2.05],[0 0])
  Auto49 : PMComponent  Tag=PSATblock  Description=Power Flow  PhysicalDomain=psatdomain  LeftPortType=p1  RightPortType=p1  LConnTagsString=__newl0  RConnTagsString=__newr0  mask(Line){p3_4_5q=[1350 400 60], p7q=1.7391, p8q=0.001, p9q=0.0495, p13_14_15q=[0.0  0.0  0.0], p16q=on}
      mask prompts: p3_4_5q "Power, Voltage and Frequency Ratings [MVA, kV, Hz]"; p7q "Primary and secondary voltage ratio [kV/kV]"; p8q "Resistance [p.u.]"; p9q "Reactance [p.u.]"; p13_14_15q "Imax, Pmax and Smax [p.u., p.u., p.u.]"; p16q "Connected"
      mask help: This block defines an auto-transformer.
      mask init:
      | [x,y] = fm_draw('circle');
      | [xq,yq] = fm_draw('quarter');
      mask CallbackString: |||||fm_block
      mask Display: plot(x,y,1.75*xq,yq,[-1 -1.3],[0 0],[1.75 2.05],[0 0])
  Auto5 : PMComponent  Tag=PSATblock  Description=Power Flow  PhysicalDomain=psatdomain  LeftPortType=p1  RightPortType=p1  LConnTagsString=__newl0  RConnTagsString=__newr0  mask(Line){p3_4_5q=[1500  765 60], p7q=1.9124, p8q=0.003, p9q=0.149, p13_14_15q=[0.0  0.0  0.0], p16q=on}
      mask prompts: p3_4_5q "Power, Voltage and Frequency Ratings [MVA, kV, Hz]"; p7q "Primary and secondary voltage ratio [kV/kV]"; p8q "Resistance [p.u.]"; p9q "Reactance [p.u.]"; p13_14_15q "Imax, Pmax and Smax [p.u., p.u., p.u.]"; p16q "Connected"
      mask help: This block defines an auto-transformer.
      mask init:
      | [x,y] = fm_draw('circle');
      | [xq,yq] = fm_draw('quarter');
      mask CallbackString: |||||fm_block
      mask Display: plot(x,y,1.75*xq,yq,[-1 -1.3],[0 0],[1.75 2.05],[0 0])
  Auto50 : PMComponent  Tag=PSATblock  Description=Power Flow  PhysicalDomain=psatdomain  LeftPortType=p1  RightPortType=p1  LConnTagsString=__newl0  RConnTagsString=__newr0  mask(Line){p3_4_5q=[300  230 60], p7q=2, p8q=0.01, p9q=0.16, p13_14_15q=[0.0  0.0  0.0], p16q=on}
      mask prompts: p3_4_5q "Power, Voltage and Frequency Ratings [MVA, kV, Hz]"; p7q "Primary and secondary voltage ratio [kV/kV]"; p8q "Resistance [p.u.]"; p9q "Reactance [p.u.]"; p13_14_15q "Imax, Pmax and Smax [p.u., p.u., p.u.]"; p16q "Connected"
      mask help: This block defines an auto-transformer.
      mask init:
      | [x,y] = fm_draw('circle');
      | [xq,yq] = fm_draw('quarter');
      mask CallbackString: |||||fm_block
      mask Display: plot(x,y,1.75*xq,yq,[-1 -1.3],[0 0],[1.75 2.05],[0 0])
  Auto56 : PMComponent  Tag=PSATblock  Description=Power Flow  PhysicalDomain=psatdomain  LeftPortType=p1  RightPortType=p1  LConnTagsString=__newl0  RConnTagsString=__newr0  mask(Line){p3_4_5q=[450 400 60], p7q=1.7391, p8q=0.01, p9q=0.18, p13_14_15q=[0.0  0.0  0.0], p16q=on}
      mask prompts: p3_4_5q "Power, Voltage and Frequency Ratings [MVA, kV, Hz]"; p7q "Primary and secondary voltage ratio [kV/kV]"; p8q "Resistance [p.u.]"; p9q "Reactance [p.u.]"; p13_14_15q "Imax, Pmax and Smax [p.u., p.u., p.u.]"; p16q "Connected"
      mask help: This block defines an auto-transformer.
      mask init:
      | [x,y] = fm_draw('circle');
      | [xq,yq] = fm_draw('quarter');
      mask CallbackString: |||||fm_block
      mask Display: plot(x,y,1.75*xq,yq,[-1 -1.3],[0 0],[1.75 2.05],[0 0])
  Auto6 : PMComponent  Tag=PSATblock  Description=Power Flow  PhysicalDomain=psatdomain  LeftPortType=p1  RightPortType=p1  LConnTagsString=__newl0  RConnTagsString=__newr0  mask(Line){p3_4_5q=[450  400 60], p7q=1.7391, p8q=0.001, p9q=0.0513, p13_14_15q=[0.0  0.0  0.0], p16q=on}
      mask prompts: p3_4_5q "Power, Voltage and Frequency Ratings [MVA, kV, Hz]"; p7q "Primary and secondary voltage ratio [kV/kV]"; p8q "Resistance [p.u.]"; p9q "Reactance [p.u.]"; p13_14_15q "Imax, Pmax and Smax [p.u., p.u., p.u.]"; p16q "Connected"
      mask help: This block defines an auto-transformer.
      mask init:
      | [x,y] = fm_draw('circle');
      | [xq,yq] = fm_draw('quarter');
      mask CallbackString: |||||fm_block
      mask Display: plot(x,y,1.75*xq,yq,[-1 -1.3],[0 0],[1.75 2.05],[0 0])
  Auto60 : PMComponent  Tag=PSATblock  Description=Power Flow  PhysicalDomain=psatdomain  LeftPortType=p1  RightPortType=p1  LConnTagsString=__newl0  RConnTagsString=__newr0  mask(Line){p3_4_5q=[333 230 60], p7q=1.6666, p8q=0.01, p9q=0.16, p13_14_15q=[0.0  0.0  0.0], p16q=on}
      mask prompts: p3_4_5q "Power, Voltage and Frequency Ratings [MVA, kV, Hz]"; p7q "Primary and secondary voltage ratio [kV/kV]"; p8q "Resistance [p.u.]"; p9q "Reactance [p.u.]"; p13_14_15q "Imax, Pmax and Smax [p.u., p.u., p.u.]"; p16q "Connected"
      mask help: This block defines an auto-transformer.
      mask init:
      | [x,y] = fm_draw('circle');
      | [xq,yq] = fm_draw('quarter');
      mask CallbackString: |||||fm_block
      mask Display: plot(x,y,1.75*xq,yq,[-1 -1.3],[0 0],[1.75 2.05],[0 0])
  Auto66 : PMComponent  Tag=PSATblock  Description=Power Flow  PhysicalDomain=psatdomain  LeftPortType=p1  RightPortType=p1  LConnTagsString=__newl0  RConnTagsString=__newr0  mask(Line){p3_4_5q=[300  400 60], p7q=1.1*400/230, p8q=0.01, p9q=0.18, p13_14_15q=[0.0  0.0  0.0], p16q=on}
      mask prompts: p3_4_5q "Power, Voltage and Frequency Ratings [MVA, kV, Hz]"; p7q "Primary and secondary voltage ratio [kV/kV]"; p8q "Resistance [p.u.]"; p9q "Reactance [p.u.]"; p13_14_15q "Imax, Pmax and Smax [p.u., p.u., p.u.]"; p16q "Connected"
      mask help: This block defines an auto-transformer.
      mask init:
      | [x,y] = fm_draw('circle');
      | [xq,yq] = fm_draw('quarter');
      mask CallbackString: |||||fm_block
      mask Display: plot(x,y,1.75*xq,yq,[-1 -1.3],[0 0],[1.75 2.05],[0 0])
  Auto7 : PMComponent  Tag=PSATblock  Description=Power Flow  PhysicalDomain=psatdomain  LeftPortType=p1  RightPortType=p1  LConnTagsString=__newl0  RConnTagsString=__newr0  mask(Line){p3_4_5q=[450  400 60], p7q=1.7391, p8q=0.001, p9q=0.0513, p13_14_15q=[0.0  0.0  0.0], p16q=on}
      mask prompts: p3_4_5q "Power, Voltage and Frequency Ratings [MVA, kV, Hz]"; p7q "Primary and secondary voltage ratio [kV/kV]"; p8q "Resistance [p.u.]"; p9q "Reactance [p.u.]"; p13_14_15q "Imax, Pmax and Smax [p.u., p.u., p.u.]"; p16q "Connected"
      mask help: This block defines an auto-transformer.
      mask init:
      | [x,y] = fm_draw('circle');
      | [xq,yq] = fm_draw('quarter');
      mask CallbackString: |||||fm_block
      mask Display: plot(x,y,1.75*xq,yq,[-1 -1.3],[0 0],[1.75 2.05],[0 0])
  Auto72 : PMComponent  Tag=PSATblock  Description=Power Flow  PhysicalDomain=psatdomain  LeftPortType=p1  RightPortType=p1  LConnTagsString=__newl0  RConnTagsString=__newr0  mask(Line){p3_4_5q=[1000 765 60], p7q=3.3256, p8q=0.01, p9q=0.21, p13_14_15q=[0.0  0.0  0.0], p16q=on}
      mask prompts: p3_4_5q "Power, Voltage and Frequency Ratings [MVA, kV, Hz]"; p7q "Primary and secondary voltage ratio [kV/kV]"; p8q "Resistance [p.u.]"; p9q "Reactance [p.u.]"; p13_14_15q "Imax, Pmax and Smax [p.u., p.u., p.u.]"; p16q "Connected"
      mask help: This block defines an auto-transformer.
      mask init:
      | [x,y] = fm_draw('circle');
      | [xq,yq] = fm_draw('quarter');
      mask CallbackString: |||||fm_block
      mask Display: plot(x,y,1.75*xq,yq,[-1 -1.3],[0 0],[1.75 2.05],[0 0])
  Auto73 : PMComponent  Tag=PSATblock  Description=Power Flow  PhysicalDomain=psatdomain  LeftPortType=p1  RightPortType=p1  LConnTagsString=__newl0  RConnTagsString=__newr0  mask(Line){p3_4_5q=[600 400 60], p7q=1.7391, p8q=0.0024, p9q=0.10, p13_14_15q=[0.0  0.0  0.0], p16q=on}
      mask prompts: p3_4_5q "Power, Voltage and Frequency Ratings [MVA, kV, Hz]"; p7q "Primary and secondary voltage ratio [kV/kV]"; p8q "Resistance [p.u.]"; p9q "Reactance [p.u.]"; p13_14_15q "Imax, Pmax and Smax [p.u., p.u., p.u.]"; p16q "Connected"
      mask help: This block defines an auto-transformer.
      mask init:
      | [x,y] = fm_draw('circle');
      | [xq,yq] = fm_draw('quarter');
      mask CallbackString: |||||fm_block
      mask Display: plot(x,y,1.75*xq,yq,[-1 -1.3],[0 0],[1.75 2.05],[0 0])
  Auto8 : PMComponent  Tag=PSATblock  Description=Power Flow  PhysicalDomain=psatdomain  LeftPortType=p1  RightPortType=p1  LConnTagsString=__newl0  RConnTagsString=__newr0  mask(Line){p3_4_5q=[300  230 60], p7q=2, p8q=0.0018, p9q=0.075, p13_14_15q=[0.0  0.0  0.0], p16q=on}
      mask prompts: p3_4_5q "Power, Voltage and Frequency Ratings [MVA, kV, Hz]"; p7q "Primary and secondary voltage ratio [kV/kV]"; p8q "Resistance [p.u.]"; p9q "Reactance [p.u.]"; p13_14_15q "Imax, Pmax and Smax [p.u., p.u., p.u.]"; p16q "Connected"
      mask help: This block defines an auto-transformer.
      mask init:
      | [x,y] = fm_draw('circle');
      | [xq,yq] = fm_draw('quarter');
      mask CallbackString: |||||fm_block
      mask Display: plot(x,y,1.75*xq,yq,[-1 -1.3],[0 0],[1.75 2.05],[0 0])
  Auto9 : PMComponent  Tag=PSATblock  Description=Power Flow  PhysicalDomain=psatdomain  LeftPortType=p1  RightPortType=p1  LConnTagsString=__newl0  RConnTagsString=__newr0  mask(Line){p3_4_5q=[450  230 60], p7q=2, p8q=0.01, p9q=0.16, p13_14_15q=[0.0  0.0  0.0], p16q=on}
      mask prompts: p3_4_5q "Power, Voltage and Frequency Ratings [MVA, kV, Hz]"; p7q "Primary and secondary voltage ratio [kV/kV]"; p8q "Resistance [p.u.]"; p9q "Reactance [p.u.]"; p13_14_15q "Imax, Pmax and Smax [p.u., p.u., p.u.]"; p16q "Connected"
      mask help: This block defines an auto-transformer.
      mask init:
      | [x,y] = fm_draw('circle');
      | [xq,yq] = fm_draw('quarter');
      mask CallbackString: |||||fm_block
      mask Display: plot(x,y,1.75*xq,yq,[-1 -1.3],[0 0],[1.75 2.05],[0 0])
  Barbacoa I 230kV : PMComponent  Tag=PSATblock  Description=Connection  PhysicalDomain=psatdomain  LeftPortType=p1  RightPortType=p1  LConnTagsString=__newl0|__newl1|__newl2  RConnTagsString=__newr0|__newr1|__newr2|__newr3  mask(Bus){in=3, out=4, p2q=230, p3_4q=[1.0002     -0.2833], p5q=1, p6q=1}
      mask prompts: in "Number of inputs:"; out "Number of outputs:"; p2q "Voltage Rating [kV]"; p3_4q "Voltage initial guess [p.u.  rad]"; p5q "Area number"; p6q "Region number"
      mask help: Bus block.
      mask init:
      | fm_inout
      settings: AttributesFormatString="|V| =  1.0061 p.u.\\n<V  = -0.0123 rad"
      mask CallbackString: ||||fm_block|
      mask Display: plot([0 1 1 0 0],[0 0 1 1 0])
  Barbacoa II 230kV : PMComponent  Tag=PSATblock  Description=Connection  PhysicalDomain=psatdomain  LeftPortType=p1  RightPortType=p1  LConnTagsString=__newl0|__newl1|__newl2|__newl3  RConnTagsString=__newr0  mask(Bus){in=4, out=1, p2q=230, p3_4q=[1.008    -0.27165], p5q=1, p6q=1}
      mask prompts: in "Number of inputs:"; out "Number of outputs:"; p2q "Voltage Rating [kV]"; p3_4q "Voltage initial guess [p.u.  rad]"; p5q "Area number"; p6q "Region number"
      mask help: Bus block.
      mask init:
      | fm_inout
      settings: AttributesFormatString="|V| =  1.0113 p.u.\\n<V  =  0.0042 rad"
      mask CallbackString: ||||fm_block|
      mask Display: plot([0 1 1 0 0],[0 0 1 1 0])
  Barbacoa II 400kV : PMComponent  Tag=PSATblock  Description=Connection  PhysicalDomain=psatdomain  LeftPortType=p1  RightPortType=p1  LConnTagsString=__newl0|__newl1  RConnTagsString=__newr0  mask(Bus){in=2, out=1, p2q=400, p3_4q=[1.0265    -0.25382], p5q=1, p6q=1}
      mask prompts: in "Number of inputs:"; out "Number of outputs:"; p2q "Voltage Rating [kV]"; p3_4q "Voltage initial guess [p.u.  rad]"; p5q "Area number"; p6q "Region number"
      mask help: Bus block.
      mask init:
      | fm_inout
      settings: AttributesFormatString="|V| =  1.0205 p.u.\\n<V  = -0.0155 rad"
      mask CallbackString: ||||fm_block|
      mask Display: plot([0 1 1 0 0],[0 0 1 1 0])
  Barinas I : PMComponent  Tag=PSATblock  Description=Connection  PhysicalDomain=psatdomain  LeftPortType=p1  RightPortType=p1  LConnTagsString=__newl0|__newl1|__newl2|__newl3|__newl4|__newl5  RConnTagsString=__newr0|__newr1|__newr2|__newr3  mask(Bus){in=6, out=4, p2q=115, p3_4q=[0.98444    -0.26004], p5q=1, p6q=1}
      mask prompts: in "Number of inputs:"; out "Number of outputs:"; p2q "Voltage Rating [kV]"; p3_4q "Voltage initial guess [p.u.  rad]"; p5q "Area number"; p6q "Region number"
      mask help: Bus block.
      mask init:
      | fm_inout
      settings: AttributesFormatString="|V| =  1.02   p.u.\\n<V  =  0.1087 rad"
      mask CallbackString: ||||fm_block|
      mask Display: plot([0 1 1 0 0],[0 0 1 1 0])
  Barinas II : PMComponent  Tag=PSATblock  Description=Connection  PhysicalDomain=psatdomain  LeftPortType=p1  RightPortType=p1  LConnTagsString=__newl0|__newl1  RConnTagsString=__newr0|__newr1  mask(Bus){in=2, out=2, p2q=115, p3_4q=[1.0023    -0.25717], p5q=1, p6q=1}
      mask prompts: in "Number of inputs:"; out "Number of outputs:"; p2q "Voltage Rating [kV]"; p3_4q "Voltage initial guess [p.u.  rad]"; p5q "Area number"; p6q "Region number"
      mask help: Bus block.
      mask init:
      | fm_inout
      settings: AttributesFormatString="|V| =  1.0216 p.u.\\n<V  =  0.1083 rad"
      mask CallbackString: ||||fm_block|
      mask Display: plot([0 1 1 0 0],[0 0 1 1 0])
  Barinas III : PMComponent  Tag=PSATblock  Description=Connection  PhysicalDomain=psatdomain  LeftPortType=p1  RightPortType=p1  LConnTagsString=__newl0|__newl1  RConnTagsString=__newr0  mask(Bus){in=2, out=1, p2q=115, p3_4q=[1.0023    -0.25717], p5q=1, p6q=1}
      mask prompts: in "Number of inputs:"; out "Number of outputs:"; p2q "Voltage Rating [kV]"; p3_4q "Voltage initial guess [p.u.  rad]"; p5q "Area number"; p6q "Region number"
      mask help: Bus block.
      mask init:
      | fm_inout
      settings: AttributesFormatString="|V| =  1.0207 p.u.\\n<V  =  0.1082 rad"
      mask CallbackString: ||||fm_block|
      mask Display: plot([0 1 1 0 0],[0 0 1 1 0])
  Barinas IV 115kV : PMComponent  Tag=PSATblock  Description=Connection  PhysicalDomain=psatdomain  LeftPortType=p1  RightPortType=p1  LConnTagsString=__newl0|__newl1|__newl2  RConnTagsString=__newr0|__newr1|__newr2|__newr3  mask(Bus){in=3, out=4, p2q=115, p3_4q=[0.98444    -0.26004], p5q=1, p6q=1}
      mask prompts: in "Number of inputs:"; out "Number of outputs:"; p2q "Voltage Rating [kV]"; p3_4q "Voltage initial guess [p.u.  rad]"; p5q "Area number"; p6q "Region number"
      mask help: Bus block.
      mask init:
      | fm_inout
      settings: AttributesFormatString="|V| =  1.0215 p.u.\\n<V  =  0.109  rad"
      mask CallbackString: ||||fm_block|
      mask Display: plot([0 1 1 0 0],[0 0 1 1 0])
  Barinas IV 230kV : PMComponent  Tag=PSATblock  Description=Connection  PhysicalDomain=psatdomain  LeftPortType=p1  RightPortType=p1  LConnTagsString=__newl0|__newl1|__newl2|__newl3|__newl4  RConnTagsString=__newr0  mask(Bus){in=5, out=1, p2q=230, p3_4q=[1.0576    -0.61106], p5q=1, p6q=1}
      mask prompts: in "Number of inputs:"; out "Number of outputs:"; p2q "Voltage Rating [kV]"; p3_4q "Voltage initial guess [p.u.  rad]"; p5q "Area number"; p6q "Region number"
      mask help: Bus block.
      mask init:
      | fm_inout
      settings: AttributesFormatString="|V| =  1.0203 p.u.\\n<V  =  0.1191 rad"
      mask CallbackString: ||||fm_block|
      mask Display: plot([0 1 1 0 0],[0 0 1 1 0])
  Boa Vista (Brasil) : PMComponent  Tag=PSATblock  Description=Connection  PhysicalDomain=psatdomain  LeftPortType=p1  RightPortType=p1  LConnTagsString=__newl0  RConnTagsString=__newr0  mask(Bus){in=1, out=1, p2q=230, p3_4q=[0.96771    -0.42846], p5q=1, p6q=1}
      mask prompts: in "Number of inputs:"; out "Number of outputs:"; p2q "Voltage Rating [kV]"; p3_4q "Voltage initial guess [p.u.  rad]"; p5q "Area number"; p6q "Region number"
      mask help: Bus block.
      mask init:
      | fm_inout
      settings: AttributesFormatString="|V| =  0.9317 p.u.\\n<V  = -0.4242 rad"
      mask CallbackString: ||||fm_block|
      mask Display: plot([0 1 1 0 0],[0 0 1 1 0])
  Boyaca 230kV : PMComponent  Tag=PSATblock  Description=Connection  PhysicalDomain=psatdomain  LeftPortType=p1  RightPortType=p1  LConnTagsString=__newl0|__newl1  RConnTagsString=__newr0  mask(Bus){in=2, out=1, p2q=230, p3_4q=[0.99306    -0.51836], p5q=1, p6q=1}
      mask prompts: in "Number of inputs:"; out "Number of outputs:"; p2q "Voltage Rating [kV]"; p3_4q "Voltage initial guess [p.u.  rad]"; p5q "Area number"; p6q "Region number"
      mask help: Bus block.
      mask init:
      | fm_inout
      settings: AttributesFormatString="|V| =  0.9941 p.u.\\n<V  = -0.2514 rad"
      mask CallbackString: ||||fm_block|
      mask Display: plot([0 1 1 0 0],[0 0 1 1 0])
  Buena Vista 115kV : PMComponent  Tag=PSATblock  Description=Connection  PhysicalDomain=psatdomain  LeftPortType=p1  RightPortType=p1  LConnTagsString=__newl0|__newl1  RConnTagsString=__newr0|__newr1|__newr2|__newr3  mask(Bus){in=2, out=4, p2q=115, p3_4q=[0.98444    -0.26004], p5q=1, p6q=1}
      mask prompts: in "Number of inputs:"; out "Number of outputs:"; p2q "Voltage Rating [kV]"; p3_4q "Voltage initial guess [p.u.  rad]"; p5q "Area number"; p6q "Region number"
      mask help: Bus block.
      mask init:
      | fm_inout
      settings: AttributesFormatString="|V| =  1.0369 p.u.\\n<V  =  0.126  rad"
      mask CallbackString: ||||fm_block|
      mask Display: plot([0 1 1 0 0],[0 0 1 1 0])
  Buena Vista 230kV : PMComponent  Tag=PSATblock  Description=Connection  PhysicalDomain=psatdomain  LeftPortType=p1  RightPortType=p1  LConnTagsString=__newl0|__newl1  RConnTagsString=__newr0|__newr1  mask(Bus){in=2, out=2, p2q=230, p3_4q=[1.0195    -0.72939], p5q=1, p6q=1}
      mask prompts: in "Number of inputs:"; out "Number of outputs:"; p2q "Voltage Rating [kV]"; p3_4q "Voltage initial guess [p.u.  rad]"; p5q "Area number"; p6q "Region number"
      mask help: Bus block.
      mask init:
      | fm_inout
      settings: AttributesFormatString="|V| =  1.0266 p.u.\\n<V  =  0.1735 rad"
      mask CallbackString: ||||fm_block|
      mask Display: plot([0 1 1 0 0],[0 0 1 1 0])
  Cabimas 230kV : PMComponent  Tag=PSATblock  Description=Connection  PhysicalDomain=psatdomain  LeftPortType=p1  RightPortType=p1  LConnTagsString=__newl0|__newl1  RConnTagsString=__newr0|__newr1  mask(Bus){in=2, out=2, p2q=230, p3_4q=[0.95441    -0.84457], p5q=1, p6q=1}
      mask prompts: in "Number of inputs:"; out "Number of outputs:"; p2q "Voltage Rating [kV]"; p3_4q "Voltage initial guess [p.u.  rad]"; p5q "Area number"; p6q "Region number"
      mask help: Bus block.
      mask init:
      | fm_inout
      settings: AttributesFormatString="|V| =  1.0002 p.u.\\n<V  =  0.1435 rad"
      mask CallbackString: ||||fm_block|
      mask Display: plot([0 1 1 0 0],[0 0 1 1 0])
  Cabudare 230kV : PMComponent  Tag=PSATblock  Description=Connection  PhysicalDomain=psatdomain  LeftPortType=p1  RightPortType=p1  LConnTagsString=__newl0  RConnTagsString=__newr0|__newr1|__newr2  mask(Bus){in=1, out=3, p2q=230, p3_4q=[0.92897    -0.59157], p5q=1, p6q=1}
      mask prompts: in "Number of inputs:"; out "Number of outputs:"; p2q "Voltage Rating [kV]"; p3_4q "Voltage initial guess [p.u.  rad]"; p5q "Area number"; p6q "Region number"
      mask help: Bus block.
      mask init:
      | fm_inout
      settings: AttributesFormatString="|V| =  0.9239 p.u.\\n<V  = -0.1915 rad"
      mask CallbackString: ||||fm_block|
      mask Display: plot([0 1 1 0 0],[0 0 1 1 0])
  Caja Seca : PMComponent  Tag=PSATblock  Description=Connection  PhysicalDomain=psatdomain  LeftPortType=p1  RightPortType=p1  LConnTagsString=__newl0  RConnTagsString=__newr0|__newr1  mask(Bus){in=1, out=2, p2q=115, p3_4q=[1.0023    -0.25717], p5q=1, p6q=1}
      mask prompts: in "Number of inputs:"; out "Number of outputs:"; p2q "Voltage Rating [kV]"; p3_4q "Voltage initial guess [p.u.  rad]"; p5q "Area number"; p6q "Region number"
      mask help: Bus block.
      mask init:
      | fm_inout
      settings: AttributesFormatString="|V| =  1.0366 p.u.\\n<V  =  0.1223 rad"
      mask CallbackString: ||||fm_block|
      mask Display: plot([0 1 1 0 0],[0 0 1 1 0])
  Calabozo 230kV : PMComponent  Tag=PSATblock  Description=Connection  PhysicalDomain=psatdomain  LeftPortType=p1  RightPortType=p1  LConnTagsString=__newl0|__newl1|__newl2  RConnTagsString=__newr0|__newr1|__newr2  mask(Bus){in=3, out=3, p2q=230, p3_4q=[0.99766    -0.53707], p5q=1, p6q=1}
      mask prompts: in "Number of inputs:"; out "Number of outputs:"; p2q "Voltage Rating [kV]"; p3_4q "Voltage initial guess [p.u.  rad]"; p5q "Area number"; p6q "Region number"
      mask help: Bus block.
      mask init:
      | fm_inout
      settings: AttributesFormatString="|V| =  1.0221 p.u.\\n<V  = -0.1592 rad"
      mask CallbackString: ||||fm_block|
      mask Display: plot([0 1 1 0 0],[0 0 1 1 0])
  Cariaco : PMComponent  Tag=PSATblock  Description=Connection  PhysicalDomain=psatdomain  LeftPortType=p1  RightPortType=p1  LConnTagsString=__newl0|__newl1  RConnTagsString=__newr0  mask(Bus){in=2, out=1, p2q=115, p3_4q=[0.99722    -0.20566], p5q=1, p6q=1}
      mask prompts: in "Number of inputs:"; out "Number of outputs:"; p2q "Voltage Rating [kV]"; p3_4q "Voltage initial guess [p.u.  rad]"; p5q "Area number"; p6q "Region number"
      mask help: Bus block.
      mask init:
      | fm_inout
      settings: AttributesFormatString="|V| =  0.9641 p.u.\\n<V  =  0.0962 rad"
      mask CallbackString: ||||fm_block|
      mask Display: plot([0 1 1 0 0],[0 0 1 1 0])
  Caruachi : PMComponent  Tag=PSATblock  Description=Connection  PhysicalDomain=psatdomain  LeftPortType=p1  RightPortType=p1  LConnTagsString=__newl0|__newl1|__newl2  RConnTagsString=__newr0  mask(Bus){in=3, out=1, p2q=400, p3_4q=[1.07   -0.020149], p5q=1, p6q=1}
      mask prompts: in "Number of inputs:"; out "Number of outputs:"; p2q "Voltage Rating [kV]"; p3_4q "Voltage initial guess [p.u.  rad]"; p5q "Area number"; p6q "Region number"
      mask help: Bus block.
      mask init:
      | fm_inout
      settings: AttributesFormatString="|V| =  1.03   p.u.\\n<V  =  0.0219 rad"
      mask CallbackString: ||||fm_block|
      mask Display: plot([0 1 1 0 0],[0 0 1 1 0])
  Casanay 115kV : PMComponent  Tag=PSATblock  Description=Connection  PhysicalDomain=psatdomain  LeftPortType=p1  RightPortType=p1  LConnTagsString=__newl0|__newl1  RConnTagsString=__newr0|__newr1|__newr2|__newr3  mask(Bus){in=2, out=4, p2q=115, p3_4q=[1.0009    -0.19751], p5q=1, p6q=1}
      mask prompts: in "Number of inputs:"; out "Number of outputs:"; p2q "Voltage Rating [kV]"; p3_4q "Voltage initial guess [p.u.  rad]"; p5q "Area number"; p6q "Region number"
      mask help: Bus block.
      mask init:
      | fm_inout
      settings: AttributesFormatString="|V| =  0.9661 p.u.\\n<V  =  0.1044 rad"
      mask CallbackString: ||||fm_block|
      mask Display: plot([0 1 1 0 0],[0 0 1 1 0])
  Casanay 230kV : PMComponent  Tag=PSATblock  Description=Connection  PhysicalDomain=psatdomain  LeftPortType=p1  RightPortType=p1  LConnTagsString=__newl0  RConnTagsString=__newr0|__newr1|__newr2|__newr3  mask(Bus){in=1, out=4, p2q=230, p3_4q=[1.0178    -0.22895], p5q=1, p6q=1}
      mask prompts: in "Number of inputs:"; out "Number of outputs:"; p2q "Voltage Rating [kV]"; p3_4q "Voltage initial guess [p.u.  rad]"; p5q "Area number"; p6q "Region number"
      mask help: Bus block.
      mask init:
      | fm_inout
      settings: AttributesFormatString="|V| =  0.9858 p.u.\\n<V  =  0.0516 rad"
      mask CallbackString: ||||fm_block|
      mask Display: plot([0 1 1 0 0],[0 0 1 1 0])
  Caña de Azucar 230kV : PMComponent  Tag=PSATblock  Description=Connection  PhysicalDomain=psatdomain  LeftPortType=p1  RightPortType=p1  LConnTagsString=__newl0|__newl1  RConnTagsString=__newr0  mask(Bus){in=2, out=1, p2q=230, p3_4q=[0.94143    -0.58376], p5q=1, p6q=1}
      mask prompts: in "Number of inputs:"; out "Number of outputs:"; p2q "Voltage Rating [kV]"; p3_4q "Voltage initial guess [p.u.  rad]"; p5q "Area number"; p6q "Region number"
      mask help: Bus block.
      mask init:
      | fm_inout
      settings: AttributesFormatString="|V| =  0.9999 p.u.\\n<V  = -0.2783 rad"
      mask CallbackString: ||||fm_block|
      mask Display: plot([0 1 1 0 0],[0 0 1 1 0])
  Cemento Andino : PMComponent  Tag=PSATblock  Description=Connection  PhysicalDomain=psatdomain  LeftPortType=p1  RightPortType=p1  LConnTagsString=__newl0  RConnTagsString=__newr0  mask(Bus){in=1, out=1, p2q=115, p3_4q=[1.0023    -0.25717], p5q=1, p6q=1}
      mask prompts: in "Number of inputs:"; out "Number of outputs:"; p2q "Voltage Rating [kV]"; p3_4q "Voltage initial guess [p.u.  rad]"; p5q "Area number"; p6q "Region number"
      mask help: Bus block.
      mask init:
      | fm_inout
      settings: AttributesFormatString="|V| =  1.0268 p.u.\\n<V  =  0.0900 rad"
      mask CallbackString: ||||fm_block|
      mask Display: plot([0 1 1 0 0],[0 0 1 1 0])
  Chicopata : PMComponent  Tag=PSATblock  Description=Connection  PhysicalDomain=psatdomain  LeftPortType=p1  RightPortType=p1  LConnTagsString=__newl0|__newl1  RConnTagsString=__newr0  mask(Bus){in=2, out=1, p2q=115, p3_4q=[1.0447   -0.081846], p5q=1, p6q=1}
      mask prompts: in "Number of inputs:"; out "Number of outputs:"; p2q "Voltage Rating [kV]"; p3_4q "Voltage initial guess [p.u.  rad]"; p5q "Area number"; p6q "Region number"
      mask help: Bus block.
      mask init:
      | fm_inout
      settings: AttributesFormatString="|V| =  1.024  p.u.\\n<V  =  0.3500 rad"
      mask CallbackString: ||||fm_block|
      mask Display: plot([0 1 1 0 0],[0 0 1 1 0])
  Ciudad Bolivar 230kV : PMComponent  Tag=PSATblock  Description=Connection  PhysicalDomain=psatdomain  LeftPortType=p1  RightPortType=p1  LConnTagsString=__newl0|__newl1  RConnTagsString=__newr0|__newr1|__newr2  mask(Bus){in=2, out=3, p2q=230, p3_4q=[1.0183    -0.23912], p5q=1, p6q=1}
      mask prompts: in "Number of inputs:"; out "Number of outputs:"; p2q "Voltage Rating [kV]"; p3_4q "Voltage initial guess [p.u.  rad]"; p5q "Area number"; p6q "Region number"
      mask help: Bus block.
      mask init:
      | fm_inout
      settings: AttributesFormatString="|V| =  0.9959 p.u.\\n<V  = -0.0787 rad"
      mask CallbackString: ||||fm_block|
      mask Display: plot([0 1 1 0 0],[0 0 1 1 0])
  Ciudad Losada 230kV : PMComponent  Tag=PSATblock  Description=Connection  PhysicalDomain=psatdomain  LeftPortType=p1  RightPortType=p1  LConnTagsString=__newl0|__newl1|__newl2|__newl3  RConnTagsString=__newr0|__newr1  mask(Bus){in=4, out=2, p2q=230, p3_4q=[0.9367    -0.47429], p5q=1, p6q=1}
      mask prompts: in "Number of inputs:"; out "Number of outputs:"; p2q "Voltage Rating [kV]"; p3_4q "Voltage initial guess [p.u.  rad]"; p5q "Area number"; p6q "Region number"
      mask help: Bus block.
      mask init:
      | fm_inout
      settings: AttributesFormatString="|V| =  1.006  p.u.\\n<V  = -0.1772 rad"
      mask CallbackString: ||||fm_block|
      mask Display: plot([0 1 1 0 0],[0 0 1 1 0])
  Ciudad Losada 400kV : PMComponent  Tag=PSATblock  Description=Connection  PhysicalDomain=psatdomain  LeftPortType=p1  RightPortType=p1  LConnTagsString=__newl0  RConnTagsString=__newr0  mask(Bus){in=1, out=1, p2q=400, p3_4q=[0.90978    -0.37531], p5q=1, p6q=1}
      mask prompts: in "Number of inputs:"; out "Number of outputs:"; p2q "Voltage Rating [kV]"; p3_4q "Voltage initial guess [p.u.  rad]"; p5q "Area number"; p6q "Region number"
      mask help: Bus block.
      mask init:
      | fm_inout
      settings: AttributesFormatString="|V| =  1.0159 p.u.\\n<V  = -0.1585 rad"
      mask CallbackString: ||||fm_block|
      mask Display: plot([0 1 1 0 0],[0 0 1 1 0])
  Convento 230kV : PMComponent  Tag=PSATblock  Description=Connection  PhysicalDomain=psatdomain  LeftPortType=p1  RightPortType=p1  LConnTagsString=__newl0|__newl1|__newl2  RConnTagsString=__newr0  mask(Bus){in=3, out=1, p2q=230, p3_4q=[0.97044    -0.53562], p5q=1, p6q=1}
      mask prompts: in "Number of inputs:"; out "Number of outputs:"; p2q "Voltage Rating [kV]"; p3_4q "Voltage initial guess [p.u.  rad]"; p5q "Area number"; p6q "Region number"
      mask help: Bus block.
      mask init:
      | fm_inout
      settings: AttributesFormatString="|V| =  0.9804 p.u.\\n<V  = -0.2644 rad"
      mask CallbackString: ||||fm_block|
      mask Display: plot([0 1 1 0 0],[0 0 1 1 0])
  Coro II : PMComponent  Tag=PSATblock  Description=Connection  PhysicalDomain=psatdomain  LeftPortType=p1  RightPortType=p1  LConnTagsString=__newl0|__newl1  RConnTagsString=__newr0|__newr1  mask(Bus){in=2, out=2, p2q=115, p3_4q=[1.02      -0.118], p5q=1, p6q=1}
      mask prompts: in "Number of inputs:"; out "Number of outputs:"; p2q "Voltage Rating [kV]"; p3_4q "Voltage initial guess [p.u.  rad]"; p5q "Area number"; p6q "Region number"
      mask help: Bus block.
      mask init:
      | fm_inout
      settings: AttributesFormatString="|V| =  1.04   p.u.\\n<V  =  0.5906 rad"
      mask CallbackString: ||||fm_block|
      mask Display: plot([0 1 1 0 0],[0 0 1 1 0])
  Cuatricentenario 138kV : PMComponent  Tag=PSATblock  Description=Connection  PhysicalDomain=psatdomain  LeftPortType=p1  RightPortType=p1  LConnTagsString=__newl0  RConnTagsString=__newr0|__newr1  mask(Bus){in=1, out=2, p2q=138, p3_4q=[1.0046    -0.90972], p5q=1, p6q=1}
      mask prompts: in "Number of inputs:"; out "Number of outputs:"; p2q "Voltage Rating [kV]"; p3_4q "Voltage initial guess [p.u.  rad]"; p5q "Area number"; p6q "Region number"
      mask help: Bus block.
      mask init:
      | fm_inout
      settings: AttributesFormatString="|V| =  0.9939 p.u.\\n<V  = -0.0296 rad"
      mask CallbackString: ||||fm_block|
      mask Display: plot([0 1 1 0 0],[0 0 1 1 0])
  Cuatricentenario 230kV : PMComponent  Tag=PSATblock  Description=Connection  PhysicalDomain=psatdomain  LeftPortType=p1  RightPortType=p1  LConnTagsString=__newl0|__newl1|__newl2|__newl3|__newl4  RConnTagsString=__newr0|__newr1  mask(Bus){in=5, out=2, p2q=230, p3_4q=[0.99316    -0.83224], p5q=1, p6q=1}
      mask prompts: in "Number of inputs:"; out "Number of outputs:"; p2q "Voltage Rating [kV]"; p3_4q "Voltage initial guess [p.u.  rad]"; p5q "Area number"; p6q "Region number"
      mask help: Bus block.
      mask init:
      | fm_inout
      settings: AttributesFormatString="|V| =  1.0282 p.u.\\n<V  = -0.0238 rad"
      mask CallbackString: ||||fm_block|
      mask Display: plot([0 1 1 0 0],[0 0 1 1 0])
  Cuatricentenario 400kV : PMComponent  Tag=PSATblock  Description=Connection  PhysicalDomain=psatdomain  LeftPortType=p1  RightPortType=p1  LConnTagsString=__newl0  RConnTagsString=__newr0|__newr1  mask(Bus){in=1, out=2, p2q=400, p3_4q=[0.96966    -0.72924], p5q=1, p6q=1}
      mask prompts: in "Number of inputs:"; out "Number of outputs:"; p2q "Voltage Rating [kV]"; p3_4q "Voltage initial guess [p.u.  rad]"; p5q "Area number"; p6q "Region number"
      mask help: Bus block.
      mask init:
      | fm_inout
      settings: AttributesFormatString="|V| =  1.0338 p.u.\\n<V  = -0.0428 rad"
      mask CallbackString: ||||fm_block|
      mask Display: plot([0 1 1 0 0],[0 0 1 1 0])
  Cuestecita (Colombia) : PMComponent  Tag=PSATblock  Description=Connection  PhysicalDomain=psatdomain  LeftPortType=p1  RightPortType=p1  LConnTagsString=__newl0  RConnTagsString=__newr0  mask(Bus){in=1, out=1, p2q=230, p3_4q=[1.0059    -0.83355], p5q=1, p6q=1}
      mask prompts: in "Number of inputs:"; out "Number of outputs:"; p2q "Voltage Rating [kV]"; p3_4q "Voltage initial guess [p.u.  rad]"; p5q "Area number"; p6q "Region number"
      mask help: Bus block.
      mask init:
      | fm_inout
      settings: AttributesFormatString="|V| =  1.0414 p.u.\\n<V  = -0.0251 rad"
      mask CallbackString: ||||fm_block|
      mask Display: plot([0 1 1 0 0],[0 0 1 1 0])
  Cumana II : PMComponent  Tag=PSATblock  Description=Connection  PhysicalDomain=psatdomain  LeftPortType=p1  RightPortType=p1  LConnTagsString=__newl0|__newl1|__newl2  RConnTagsString=__newr0|__newr1|__newr2|__newr3  mask(Bus){in=3, out=4, p2q=115, p3_4q=[0.98444    -0.26004], p5q=1, p6q=1}
      mask prompts: in "Number of inputs:"; out "Number of outputs:"; p2q "Voltage Rating [kV]"; p3_4q "Voltage initial guess [p.u.  rad]"; p5q "Area number"; p6q "Region number"
      mask help: Bus block.
      mask init:
      | fm_inout
      settings: AttributesFormatString="|V| =  0.9704 p.u.\\n<V  =  0.0459 rad"
      mask CallbackString: ||||fm_block|
      mask Display: plot([0 1 1 0 0],[0 0 1 1 0])
  Cumana III : PMComponent  Tag=PSATblock  Description=Connection  PhysicalDomain=psatdomain  LeftPortType=p1  RightPortType=p1  LConnTagsString=__newl0|__newl1  RConnTagsString=__newr0  mask(Bus){in=2, out=1, p2q=115, p3_4q=[0.98025    -0.26446], p5q=1, p6q=1}
      mask prompts: in "Number of inputs:"; out "Number of outputs:"; p2q "Voltage Rating [kV]"; p3_4q "Voltage initial guess [p.u.  rad]"; p5q "Area number"; p6q "Region number"
      mask help: Bus block.
      mask init:
      | fm_inout
      settings: AttributesFormatString="|V| =  0.9659 p.u.\\n<V  =  0.0410 rad"
      mask CallbackString: ||||fm_block|
      mask Display: plot([0 1 1 0 0],[0 0 1 1 0])
  Ejido : PMComponent  Tag=PSATblock  Description=Connection  PhysicalDomain=psatdomain  LeftPortType=p1  RightPortType=p1  LConnTagsString=__newl0  RConnTagsString=__newr0|__newr1  mask(Bus){in=1, out=2, p2q=115, p3_4q=[1.0023    -0.25717], p5q=1, p6q=1}
      mask prompts: in "Number of inputs:"; out "Number of outputs:"; p2q "Voltage Rating [kV]"; p3_4q "Voltage initial guess [p.u.  rad]"; p5q "Area number"; p6q "Region number"
      mask help: Bus block.
      mask init:
      | fm_inout
      settings: AttributesFormatString="|V| =  0.9589 p.u.\\n<V  =  0.2596 rad"
      mask CallbackString: ||||fm_block|
      mask Display: plot([0 1 1 0 0],[0 0 1 1 0])
  El Callao II 400kV : PMComponent  Tag=PSATblock  Description=Connection  PhysicalDomain=psatdomain  LeftPortType=p1  RightPortType=p1  LConnTagsString=__newl0  RConnTagsString=__newr0|__newr1  mask(Bus){in=1, out=2, p2q=400, p3_4q=[1.1192    -0.12256], p5q=1, p6q=1}
      mask prompts: in "Number of inputs:"; out "Number of outputs:"; p2q "Voltage Rating [kV]"; p3_4q "Voltage initial guess [p.u.  rad]"; p5q "Area number"; p6q "Region number"
      mask help: Bus block.
      mask init:
      | fm_inout
      settings: AttributesFormatString="|V| =  1.0718 p.u.\\n<V  = -0.0883 rad"
      mask CallbackString: ||||fm_block|
      mask Display: plot([0 1 1 0 0],[0 0 1 1 0])
  El Corozo 115kV : PMComponent  Tag=PSATblock  Description=Connection  PhysicalDomain=psatdomain  LeftPortType=p1  RightPortType=p1  LConnTagsString=__newl0|__newl1|__newl2|__newl3  RConnTagsString=__newr0|__newr1|__newr2|__newr3|__newr4  mask(Bus){in=4, out=5, p2q=115, p3_4q=[0.98444    -0.26004], p5q=1, p6q=1}
      mask prompts: in "Number of inputs:"; out "Number of outputs:"; p2q "Voltage Rating [kV]"; p3_4q "Voltage initial guess [p.u.  rad]"; p5q "Area number"; p6q "Region number"
      mask help: Bus block.
      mask init:
      | fm_inout
      settings: AttributesFormatString="|V| =  1.0161 p.u.\\n<V  =  0.4604 rad"
      mask CallbackString: ||||fm_block|
      mask Display: plot([0 1 1 0 0],[0 0 1 1 0])
  El Corozo 230kV : PMComponent  Tag=PSATblock  Description=Connection  PhysicalDomain=psatdomain  LeftPortType=p1  RightPortType=p1  LConnTagsString=__newl0|__newl1  RConnTagsString=__newr0|__newr1|__newr2|__newr3  mask(Bus){in=2, out=4, p2q=230, p3_4q=[1.0561    -0.68744], p5q=1, p6q=1}
      mask prompts: in "Number of inputs:"; out "Number of outputs:"; p2q "Voltage Rating [kV]"; p3_4q "Voltage initial guess [p.u.  rad]"; p5q "Area number"; p6q "Region number"
      mask help: Bus block.
      mask init:
      | fm_inout
      settings: AttributesFormatString="|V| =  1.0609 p.u.\\n<V  =  0.5313 rad"
      mask CallbackString: ||||fm_block|
      mask Display: plot([0 1 1 0 0],[0 0 1 1 0])
  El Indio 230kV : PMComponent  Tag=PSATblock  Description=Connection  PhysicalDomain=psatdomain  LeftPortType=p1  RightPortType=p1  LConnTagsString=__newl0|__newl1|__newl2  RConnTagsString=__newr0|__newr1|__newr2  mask(Bus){in=3, out=3, p2q=230, p3_4q=[1.0055    -0.23512], p5q=1, p6q=1}
      mask prompts: in "Number of inputs:"; out "Number of outputs:"; p2q "Voltage Rating [kV]"; p3_4q "Voltage initial guess [p.u.  rad]"; p5q "Area number"; p6q "Region number"
      mask help: Bus block.
      mask init:
      | fm_inout
      settings: AttributesFormatString="|V| =  0.9786 p.u.\\n<V  = -0.0658 rad"
      mask CallbackString: ||||fm_block|
      mask Display: plot([0 1 1 0 0],[0 0 1 1 0])
  El Playon : PMComponent  Tag=PSATblock  Description=Connection  PhysicalDomain=psatdomain  LeftPortType=p1  RightPortType=p1  LConnTagsString=__newl0|__newl1  RConnTagsString=__newr0  mask(Bus){in=2, out=1, p2q=115, p3_4q=[1.0023    -0.25717], p5q=1, p6q=1}
      mask prompts: in "Number of inputs:"; out "Number of outputs:"; p2q "Voltage Rating [kV]"; p3_4q "Voltage initial guess [p.u.  rad]"; p5q "Area number"; p6q "Region number"
      mask help: Bus block.
      mask init:
      | fm_inout
      settings: AttributesFormatString="|V| =  0.8341 p.u.\\n<V  = -0.2004 rad"
      mask CallbackString: ||||fm_block|
      mask Display: plot([0 1 1 0 0],[0 0 1 1 0])
  El Rincon 138kV : PMComponent  Tag=PSATblock  Description=Connection  PhysicalDomain=psatdomain  LeftPortType=p1  RightPortType=p1  LConnTagsString=__newl0|__newl1  RConnTagsString=__newr0|__newr1|__newr2|__newr3|__newr4  mask(Bus){in=2, out=5, p2q=138, p3_4q=[1.0573    -0.90473], p5q=1, p6q=1}
      mask prompts: in "Number of inputs:"; out "Number of outputs:"; p2q "Voltage Rating [kV]"; p3_4q "Voltage initial guess [p.u.  rad]"; p5q "Area number"; p6q "Region number"
      mask help: Bus block.
      mask init:
      | fm_inout
      settings: AttributesFormatString="|V| =  1.0254 p.u.\\n<V  =  0.0623 rad"
      mask CallbackString: ||||fm_block|
      mask Display: plot([0 1 1 0 0],[0 0 1 1 0])
  El Rincon 230kV : PMComponent  Tag=PSATblock  Description=Connection  PhysicalDomain=psatdomain  LeftPortType=p1  RightPortType=p1  LConnTagsString=__newl0  RConnTagsString=__newr0  mask(Bus){in=1, out=1, p2q=230, p3_4q=[1.0067    -0.85005], p5q=1, p6q=1}
      mask prompts: in "Number of inputs:"; out "Number of outputs:"; p2q "Voltage Rating [kV]"; p3_4q "Voltage initial guess [p.u.  rad]"; p5q "Area number"; p6q "Region number"
      mask help: Bus block.
      mask init:
      | fm_inout
      settings: AttributesFormatString="|V| =  1.0276 p.u.\\n<V  = -0.0007 rad"
      mask CallbackString: ||||fm_block|
      mask Display: plot([0 1 1 0 0],[0 0 1 1 0])
  El Tablazo 230kV : PMComponent  Tag=PSATblock  Description=Connection  PhysicalDomain=psatdomain  LeftPortType=p1  RightPortType=p1  LConnTagsString=__newl0|__newl1|__newl2|__newl3|__newl4  RConnTagsString=__newr0|__newr1  mask(Bus){in=5, out=2, p2q=230, p3_4q=[0.98193    -0.81876], p5q=1, p6q=1}
      mask prompts: in "Number of inputs:"; out "Number of outputs:"; p2q "Voltage Rating [kV]"; p3_4q "Voltage initial guess [p.u.  rad]"; p5q "Area number"; p6q "Region number"
      mask help: Bus block.
      mask init:
      | fm_inout
      settings: AttributesFormatString="|V| =  1.0269 p.u.\\n<V  = -0.0330 rad"
      mask CallbackString: ||||fm_block|
      mask Display: plot([0 1 1 0 0],[0 0 1 1 0])
  El Tablazo 400kV : PMComponent  Tag=PSATblock  Description=Connection  PhysicalDomain=psatdomain  LeftPortType=p1  RightPortType=p1  LConnTagsString=__newl0|__newl1|__newl2  RConnTagsString=__newr0|__newr1|__newr2|__newr3  mask(Bus){in=3, out=4, p2q=400, p3_4q=[0.96726    -0.71909], p5q=1, p6q=1}
      mask prompts: in "Number of inputs:"; out "Number of outputs:"; p2q "Voltage Rating [kV]"; p3_4q "Voltage initial guess [p.u.  rad]"; p5q "Area number"; p6q "Region number"
      mask help: Bus block.
      mask init:
      | fm_inout
      settings: AttributesFormatString="|V| =  1.033  p.u.\\n<V  = -0.0447 rad"
      mask CallbackString: ||||fm_block|
      mask Display: plot([0 1 1 0 0],[0 0 1 1 0])
  El Tigre 230kV : PMComponent  Tag=PSATblock  Description=Connection  PhysicalDomain=psatdomain  LeftPortType=p1  RightPortType=p1  LConnTagsString=__newl0|__newl1|__newl2|__newl3|__newl4|__newl5  RConnTagsString=__newr0|__newr1|__newr2|__newr3  mask(Bus){in=6, out=4, p2q=230, p3_4q=[0.975    -0.21147], p5q=1, p6q=1}
      mask prompts: in "Number of inputs:"; out "Number of outputs:"; p2q "Voltage Rating [kV]"; p3_4q "Voltage initial guess [p.u.  rad]"; p5q "Area number"; p6q "Region number"
      mask help: Bus block.
      mask init:
      | fm_inout
      settings: AttributesFormatString="|V| =  0.9955 p.u.\\n<V  = -0.0312 rad"
      mask CallbackString: ||||fm_block|
      mask Display: plot([0 1 1 0 0],[0 0 1 1 0])
  El Tigre 400kV : PMComponent  Tag=PSATblock  Description=Connection  PhysicalDomain=psatdomain  LeftPortType=p1  RightPortType=p1  LConnTagsString=__newl0|__newl1|__newl2|__newl3|__newl4  RConnTagsString=__newr0|__newr1|__newr2|__newr3  mask(Bus){in=5, out=4, p2q=400, p3_4q=[1.0506    -0.17198], p5q=1, p6q=1}
      mask prompts: in "Number of inputs:"; out "Number of outputs:"; p2q "Voltage Rating [kV]"; p3_4q "Voltage initial guess [p.u.  rad]"; p5q "Area number"; p6q "Region number"
      mask help: Bus block.
      mask init:
      | fm_inout
      settings: AttributesFormatString="|V| =  1.0229 p.u.\\n<V  = -0.0220 rad"
      mask CallbackString: ||||fm_block|
      mask Display: plot([0 1 1 0 0],[0 0 1 1 0])
  El Torereno : PMComponent  Tag=PSATblock  Description=Connection  PhysicalDomain=psatdomain  LeftPortType=p1  RightPortType=p1  LConnTagsString=__newl0|__newl1  RConnTagsString=__newr0|__newr1  mask(Bus){in=2, out=2, p2q=115, p3_4q=[1.0023    -0.25717], p5q=1, p6q=1}
      mask prompts: in "Number of inputs:"; out "Number of outputs:"; p2q "Voltage Rating [kV]"; p3_4q "Voltage initial guess [p.u.  rad]"; p5q "Area number"; p6q "Region number"
      mask help: Bus block.
      mask init:
      | fm_inout
      settings: AttributesFormatString="|V| =  1.0305 p.u.\\n<V  =  0.1020 rad"
      mask CallbackString: ||||fm_block|
      mask Display: plot([0 1 1 0 0],[0 0 1 1 0])
  El Vigia : PMComponent  Tag=PSATblock  Description=Connection  PhysicalDomain=psatdomain  LeftPortType=p1  RightPortType=p1  LConnTagsString=__newl0|__newl1  RConnTagsString=__newr0|__newr1|__newr2|__newr3  mask(Bus){in=2, out=4, p2q=115, p3_4q=[0.98444    -0.26004], p5q=1, p6q=1}
      mask prompts: in "Number of inputs:"; out "Number of outputs:"; p2q "Voltage Rating [kV]"; p3_4q "Voltage initial guess [p.u.  rad]"; p5q "Area number"; p6q "Region number"
      mask help: Bus block.
      mask init:
      | fm_inout
      settings: AttributesFormatString="|V| =  1.003  p.u.\\n<V  =  0.3995 rad"
      mask CallbackString: ||||fm_block|
      mask Display: plot([0 1 1 0 0],[0 0 1 1 0])
  El Vigia II 115kV : PMComponent  Tag=PSATblock  Description=Connection  PhysicalDomain=psatdomain  LeftPortType=p1  RightPortType=p1  LConnTagsString=__newl0|__newl1|__newl2  RConnTagsString=__newr0  mask(Bus){in=3, out=1, p2q=115, p3_4q=[0.98444    -0.26004], p5q=1, p6q=1}
      mask prompts: in "Number of inputs:"; out "Number of outputs:"; p2q "Voltage Rating [kV]"; p3_4q "Voltage initial guess [p.u.  rad]"; p5q "Area number"; p6q "Region number"
      mask help: Bus block.
      mask init:
      | fm_inout
      settings: AttributesFormatString="|V| =  1.0099 p.u.\\n<V  =  0.4166 rad"
      mask CallbackString: ||||fm_block|
      mask Display: plot([0 1 1 0 0],[0 0 1 1 0])
  El Vigia II 230kV : PMComponent  Tag=PSATblock  Description=Connection  PhysicalDomain=psatdomain  LeftPortType=p1  RightPortType=p1  LConnTagsString=__newl0|__newl1  RConnTagsString=__newr0|__newr1  mask(Bus){in=2, out=2, p2q=230, p3_4q=[1.0419    -0.70804], p5q=1, p6q=1}
      mask prompts: in "Number of inputs:"; out "Number of outputs:"; p2q "Voltage Rating [kV]"; p3_4q "Voltage initial guess [p.u.  rad]"; p5q "Area number"; p6q "Region number"
      mask help: Bus block.
      mask init:
      | fm_inout
      settings: AttributesFormatString="|V| =  1.019  p.u.\\n<V  =  0.4194 rad"
      mask CallbackString: ||||fm_block|
      mask Display: plot([0 1 1 0 0],[0 0 1 1 0])
  Elorza : PMComponent  Tag=PSATblock  Description=Connection  PhysicalDomain=psatdomain  LeftPortType=p1  RightPortType=p1  LConnTagsString=__newl0  RConnTagsString=__newr0|__newr1  mask(Bus){in=1, out=2, p2q=115, p3_4q=[1.0023    -0.25717], p5q=1, p6q=1}
      mask prompts: in "Number of inputs:"; out "Number of outputs:"; p2q "Voltage Rating [kV]"; p3_4q "Voltage initial guess [p.u.  rad]"; p5q "Area number"; p6q "Region number"
      mask help: Bus block.
      mask init:
      | fm_inout
      settings: AttributesFormatString="|V| =  0.9801 p.u.\\n<V  =  0.4720 rad"
      mask CallbackString: ||||fm_block|
      mask Display: plot([0 1 1 0 0],[0 0 1 1 0])
  Furrial 230kV : PMComponent  Tag=PSATblock  Description=Connection  PhysicalDomain=psatdomain  LeftPortType=p1  RightPortType=p1  LConnTagsString=__newl0|__newl1  RConnTagsString=__newr0|__newr1|__newr2  mask(Bus){in=2, out=3, p2q=230, p3_4q=[1.0017     -0.2328], p5q=1, p6q=1}
      mask prompts: in "Number of inputs:"; out "Number of outputs:"; p2q "Voltage Rating [kV]"; p3_4q "Voltage initial guess [p.u.  rad]"; p5q "Area number"; p6q "Region number"
      mask help: Bus block.
      mask init:
      | fm_inout
      settings: AttributesFormatString="|V| =  0.9790 p.u.\\n<V  = -0.0949 rad"
      mask CallbackString: ||||fm_block|
      mask Display: plot([0 1 1 0 0],[0 0 1 1 0])
  Furrial 400kV : PMComponent  Tag=PSATblock  Description=Connection  PhysicalDomain=psatdomain  LeftPortType=p1  RightPortType=p1  LConnTagsString=__newl0|__newl1  RConnTagsString=__newr0|__newr1  mask(Bus){in=2, out=2, p2q=400, p3_4q=[0.99372    -0.23808], p5q=1, p6q=1}
      mask prompts: in "Number of inputs:"; out "Number of outputs:"; p2q "Voltage Rating [kV]"; p3_4q "Voltage initial guess [p.u.  rad]"; p5q "Area number"; p6q "Region number"
      mask help: Bus block.
      mask init:
      | fm_inout
      settings: AttributesFormatString="|V| =  0.9763 p.u.\\n<V  = -0.1443 rad"
      mask CallbackString: ||||fm_block|
      mask Display: plot([0 1 1 0 0],[0 0 1 1 0])
  Gen. Anz 2012-1 : PMComponent  Tag=PSATblock  Description=Connection  PhysicalDomain=psatdomain  LeftPortType=p1  RightPortType=p1  LConnTagsString=__newl0  RConnTagsString=__newr0  mask(Bus){in=1, out=1, p2q=400, p3_4q=[1 0], p5q=1, p6q=1}
      mask prompts: in "Number of inputs:"; out "Number of outputs:"; p2q "Voltage Rating [kV]"; p3_4q "Voltage initial guess [p.u.  rad]"; p5q "Area number"; p6q "Region number"
      mask help: Bus block.
      mask init:
      | fm_inout
      settings: AttributesFormatString="|V| =  1.02   p.u.\\n<V  = -0.0248 rad"
      mask CallbackString: ||||fm_block|
      mask Display: plot([0 1 1 0 0],[0 0 1 1 0])
  Gen. Anz 2012-2 : PMComponent  Tag=PSATblock  Description=Connection  PhysicalDomain=psatdomain  LeftPortType=p1  RightPortType=p1  LConnTagsString=__newl0  RConnTagsString=__newr0  mask(Bus){in=1, out=1, p2q=400, p3_4q=[1 0], p5q=1, p6q=1}
      mask prompts: in "Number of inputs:"; out "Number of outputs:"; p2q "Voltage Rating [kV]"; p3_4q "Voltage initial guess [p.u.  rad]"; p5q "Area number"; p6q "Region number"
      mask help: Bus block.
      mask init:
      | fm_inout
      settings: AttributesFormatString="|V| =  1.02   p.u.\\n<V  = -0.0172 rad"
      mask CallbackString: ||||fm_block|
      mask Display: plot([0 1 1 0 0],[0 0 1 1 0])
  Gen. Guarico 2012 : PMComponent  Tag=PSATblock  Description=Connection  PhysicalDomain=psatdomain  LeftPortType=p1  RightPortType=p1  LConnTagsString=__newl0  RConnTagsString=__newr0  mask(Bus){in=1, out=1, p2q=230, p3_4q=[1.0021    -0.55915], p5q=1, p6q=1}
      mask prompts: in "Number of inputs:"; out "Number of outputs:"; p2q "Voltage Rating [kV]"; p3_4q "Voltage initial guess [p.u.  rad]"; p5q "Area number"; p6q "Region number"
      mask help: Bus block.
      mask init:
      | fm_inout
      settings: AttributesFormatString="|V| =  1.02   p.u.\\n<V  = -0.1496 rad"
      mask CallbackString: ||||fm_block|
      mask Display: plot([0 1 1 0 0],[0 0 1 1 0])
  Gen. Miranda 2012 : PMComponent  Tag=PSATblock  Description=Connection  PhysicalDomain=psatdomain  LeftPortType=p1  RightPortType=p1  LConnTagsString=__newl0  RConnTagsString=__newr0  mask(Bus){in=1, out=1, p2q=230, p3_4q=[1 0], p5q=1, p6q=1}
      mask prompts: in "Number of inputs:"; out "Number of outputs:"; p2q "Voltage Rating [kV]"; p3_4q "Voltage initial guess [p.u.  rad]"; p5q "Area number"; p6q "Region number"
      mask help: Bus block.
      mask init:
      | fm_inout
      settings: AttributesFormatString="|V| =  1.02   p.u.\\n<V  = -0.1307 rad"
      mask CallbackString: ||||fm_block|
      mask Display: plot([0 1 1 0 0],[0 0 1 1 0])
  Gen. Zulia 2012 : PMComponent  Tag=PSATblock  Description=Connection  PhysicalDomain=psatdomain  LeftPortType=p1  RightPortType=p1  LConnTagsString=__newl0  RConnTagsString=__newr0  mask(Bus){in=1, out=1, p2q=230, p3_4q=[1 0], p5q=1, p6q=1}
      mask prompts: in "Number of inputs:"; out "Number of outputs:"; p2q "Voltage Rating [kV]"; p3_4q "Voltage initial guess [p.u.  rad]"; p5q "Area number"; p6q "Region number"
      mask help: Bus block.
      mask init:
      | fm_inout
      settings: AttributesFormatString="|V| =  1.04   p.u.\\n<V  =  0.4457 rad"
      mask CallbackString: ||||fm_block|
      mask Display: plot([0 1 1 0 0],[0 0 1 1 0])
  Guanare : PMComponent  Tag=PSATblock  Description=Connection  PhysicalDomain=psatdomain  LeftPortType=p1  RightPortType=p1  LConnTagsString=__newl0|__newl1|__newl2  RConnTagsString=__newr0|__newr1|__newr2  mask(Bus){in=3, out=3, p2q=115, p3_4q=[0.98444    -0.26004], p5q=1, p6q=1}
      mask prompts: in "Number of inputs:"; out "Number of outputs:"; p2q "Voltage Rating [kV]"; p3_4q "Voltage initial guess [p.u.  rad]"; p5q "Area number"; p6q "Region number"
      mask help: Bus block.
      mask init:
      | fm_inout
      settings: AttributesFormatString="|V| =  0.9819 p.u.\\n<V  =  0.0254 rad"
      mask CallbackString: ||||fm_block|
      mask Display: plot([0 1 1 0 0],[0 0 1 1 0])
  Guanta II 115kV : PMComponent  Tag=PSATblock  Description=Connection  PhysicalDomain=psatdomain  LeftPortType=p1  RightPortType=p1  LConnTagsString=__newl0|__newl1  RConnTagsString=__newr0  mask(Bus){in=2, out=1, p2q=115, p3_4q=[1.0023    -0.25717], p5q=1, p6q=1}
      mask prompts: in "Number of inputs:"; out "Number of outputs:"; p2q "Voltage Rating [kV]"; p3_4q "Voltage initial guess [p.u.  rad]"; p5q "Area number"; p6q "Region number"
      mask help: Bus block.
      mask init:
      | fm_inout
      settings: AttributesFormatString="|V| =  0.9982 p.u.\\n<V  =  0.0533 rad"
      mask CallbackString: ||||fm_block|
      mask Display: plot([0 1 1 0 0],[0 0 1 1 0])
  Guanta II 230kV : PMComponent  Tag=PSATblock  Description=Connection  PhysicalDomain=psatdomain  LeftPortType=p1  RightPortType=p1  LConnTagsString=__newl0|__newl1|__newl2|__newl3  RConnTagsString=__newr0|__newr1|__newr2|__newr3  mask(Bus){in=4, out=4, p2q=230, p3_4q=[1.02    -0.24902], p5q=1, p6q=1}
      mask prompts: in "Number of inputs:"; out "Number of outputs:"; p2q "Voltage Rating [kV]"; p3_4q "Voltage initial guess [p.u.  rad]"; p5q "Area number"; p6q "Region number"
      mask help: Bus block.
      mask init:
      | fm_inout
      settings: AttributesFormatString="|V| =  1.02   p.u.\\n<V  =  0.0654 rad"
      mask CallbackString: ||||fm_block|
      mask Display: plot([0 1 1 0 0],[0 0 1 1 0])
  Guasdualito : PMComponent  Tag=PSATblock  Description=Connection  PhysicalDomain=psatdomain  LeftPortType=p1  RightPortType=p1  LConnTagsString=__newl0|__newl1|__newl2  RConnTagsString=__newr0|__newr1  mask(Bus){in=3, out=2, p2q=115, p3_4q=[1.0023    -0.25717], p5q=1, p6q=1}
      mask prompts: in "Number of inputs:"; out "Number of outputs:"; p2q "Voltage Rating [kV]"; p3_4q "Voltage initial guess [p.u.  rad]"; p5q "Area number"; p6q "Region number"
      mask help: Bus block.
      mask init:
      | fm_inout
      settings: AttributesFormatString="|V| =  0.9812 p.u.\\n<V  =  0.4730 rad"
      mask CallbackString: ||||fm_block|
      mask Display: plot([0 1 1 0 0],[0 0 1 1 0])
  Guayana A : PMComponent  Tag=PSATblock  Description=Connection  PhysicalDomain=psatdomain  LeftPortType=p1  RightPortType=p1  LConnTagsString=__newl0|__newl1|__newl2|__newl3  RConnTagsString=__newr0|__newr1  mask(Bus){in=4, out=2, p2q=230, p3_4q=[1.07    -0.19263], p5q=1, p6q=1}
      mask prompts: in "Number of inputs:"; out "Number of outputs:"; p2q "Voltage Rating [kV]"; p3_4q "Voltage initial guess [p.u.  rad]"; p5q "Area number"; p6q "Region number"
      mask help: Bus block.
      mask init:
      | fm_inout
      settings: AttributesFormatString="|V| =  1.03   p.u.\\n<V  = -0.0346 rad"
      mask CallbackString: ||||fm_block|
      mask Display: plot([0 1 1 0 0],[0 0 1 1 0])
  Guayana B : PMComponent  Tag=PSATblock  Description=Connection  PhysicalDomain=psatdomain  LeftPortType=p1  RightPortType=p1  LConnTagsString=__newl0|__newl1|__newl2|__newl3  RConnTagsString=__newr0|__newr1  mask(Bus){in=4, out=2, p2q=400, p3_4q=[1.0142    -0.15088], p5q=1, p6q=1}
      mask prompts: in "Number of inputs:"; out "Number of outputs:"; p2q "Voltage Rating [kV]"; p3_4q "Voltage initial guess [p.u.  rad]"; p5q "Area number"; p6q "Region number"
      mask help: Bus block.
      mask init:
      | fm_inout
      settings: AttributesFormatString="|V| =  1.0012 p.u.\\n<V  = -0.1147 rad"
      mask CallbackString: ||||fm_block|
      mask Display: plot([0 1 1 0 0],[0 0 1 1 0])
  Guri 230kV : PMComponent  Tag=PSATblock  Description=Connection  PhysicalDomain=psatdomain  LeftPortType=p1  RightPortType=p1  LConnTagsString=__newl0|__newl1|__newl2  RConnTagsString=__newr0  mask(Bus){in=3, out=1, p2q=230, p3_4q=[1.0719    -0.13773], p5q=1, p6q=1}
      mask prompts: in "Number of inputs:"; out "Number of outputs:"; p2q "Voltage Rating [kV]"; p3_4q "Voltage initial guess [p.u.  rad]"; p5q "Area number"; p6q "Region number"
      mask help: Bus block.
      mask init:
      | fm_inout
      settings: AttributesFormatString="|V| =  1.04   p.u.\\n<V  =  0.0223 rad"
      mask CallbackString: ||||fm_block|
      mask Display: plot([0 1 1 0 0],[0 0 1 1 0])
  Guri 400kV A : PMComponent  Tag=PSATblock  Description=Connection  PhysicalDomain=psatdomain  LeftPortType=p1  RightPortType=p1  LConnTagsString=__newl0|__newl1|__newl2|__newl3|__newl4|__newl5  RConnTagsString=__newr0|__newr1  mask(Bus){in=6, out=2, p2q=400, p3_4q=[1.07    -0.05981], p5q=1, p6q=1}
      mask prompts: in "Number of inputs:"; out "Number of outputs:"; p2q "Voltage Rating [kV]"; p3_4q "Voltage initial guess [p.u.  rad]"; p5q "Area number"; p6q "Region number"
      mask help: Bus block.
      mask init:
      | fm_inout
      settings: AttributesFormatString="|V| =  1.04   p.u.\\n<V  =  0.0088 rad"
      mask CallbackString: ||||fm_block|
      mask Display: plot([0 1 1 0 0],[0 0 1 1 0])
  Guri 400kV B : PMComponent  Tag=PSATblock  Description=Connection  PhysicalDomain=psatdomain  LeftPortType=p1  RightPortType=p1  LConnTagsString=__newl0|__newl1|__newl2|__newl3  RConnTagsString=__newr0|__newr1|__newr2  mask(Bus){in=4, out=3, p2q=400, p3_4q=[1.0552   -0.050057], p5q=1, p6q=1}
      mask prompts: in "Number of inputs:"; out "Number of outputs:"; p2q "Voltage Rating [kV]"; p3_4q "Voltage initial guess [p.u.  rad]"; p5q "Area number"; p6q "Region number"
      mask help: Bus block.
      mask init:
      | fm_inout
      settings: AttributesFormatString="|V| =  1.1174 p.u.\\n<V  = -0.0223 rad"
      mask CallbackString: ||||fm_block|
      mask Display: plot([0 1 1 0 0],[0 0 1 1 0])
  Guri 765kV : PMComponent  Tag=PSATblock  Description=Connection  PhysicalDomain=psatdomain  LeftPortType=p1  RightPortType=p1  LConnTagsString=__newl0|__newl1|__newl2|__newl3|__newl4|__newl5  RConnTagsString=__newr0|__newr1|__newr2  mask(Bus){in=6, out=3, p2q=765, p3_4q=[1.07           0], p5q=1, p6q=1}
      mask prompts: in "Number of inputs:"; out "Number of outputs:"; p2q "Voltage Rating [kV]"; p3_4q "Voltage initial guess [p.u.  rad]"; p5q "Area number"; p6q "Region number"
      mask help: Bus block.
      mask init:
      | fm_inout
      settings: AttributesFormatString="|V| =  1.04   p.u.\\n<V  =  0      rad"
      mask CallbackString: ||||fm_block|
      mask Display: plot([0 1 1 0 0],[0 0 1 1 0])
  Isiro 115kV : PMComponent  Tag=PSATblock  Description=Connection  PhysicalDomain=psatdomain  LeftPortType=p1  RightPortType=p1  LConnTagsString=__newl0|__newl1|__newl2|__newl3  RConnTagsString=__newr0  mask(Bus){in=4, out=1, p2q=115, p3_4q=[0.95525    -0.20379], p5q=1, p6q=1}
      mask prompts: in "Number of inputs:"; out "Number of outputs:"; p2q "Voltage Rating [kV]"; p3_4q "Voltage initial guess [p.u.  rad]"; p5q "Area number"; p6q "Region number"
      mask help: Bus block.
      mask init:
      | fm_inout
      settings: AttributesFormatString="|V| =  0.9617 p.u.\\n<V  =  0.5120 rad"
      mask CallbackString: ||||fm_block|
      mask Display: plot([0 1 1 0 0],[0 0 1 1 0])
  Isiro 230kV : PMComponent  Tag=PSATblock  Description=Connection  PhysicalDomain=psatdomain  LeftPortType=p1  RightPortType=p1  LConnTagsString=__newl0|__newl1  RConnTagsString=__newr0|__newr1  mask(Bus){in=2, out=2, p2q=230, p3_4q=[0.97836    -0.32408], p5q=1, p6q=1}
      mask prompts: in "Number of inputs:"; out "Number of outputs:"; p2q "Voltage Rating [kV]"; p3_4q "Voltage initial guess [p.u.  rad]"; p5q "Area number"; p6q "Region number"
      mask help: Bus block.
      mask init:
      | fm_inout
      settings: AttributesFormatString="|V| =  0.9437 p.u.\\n<V  =  0.2926 rad"
      mask CallbackString: ||||fm_block|
      mask Display: plot([0 1 1 0 0],[0 0 1 1 0])
  Jose 400kV : PMComponent  Tag=PSATblock  Description=Connection  PhysicalDomain=psatdomain  LeftPortType=p1  RightPortType=p1  LConnTagsString=__newl0|__newl1  RConnTagsString=__newr0|__newr1|__newr2  mask(Bus){in=2, out=3, p2q=400, p3_4q=[1.0223    -0.26866], p5q=1, p6q=1}
      mask prompts: in "Number of inputs:"; out "Number of outputs:"; p2q "Voltage Rating [kV]"; p3_4q "Voltage initial guess [p.u.  rad]"; p5q "Area number"; p6q "Region number"
      mask help: Bus block.
      mask init:
      | fm_inout
      settings: AttributesFormatString="|V| =  1.0197 p.u.\\n<V  = -0.0292 rad"
      mask CallbackString: ||||fm_block|
      mask Display: plot([0 1 1 0 0],[0 0 1 1 0])
  Junquito 230kV : PMComponent  Tag=PSATblock  Description=Connection  PhysicalDomain=psatdomain  LeftPortType=p1  RightPortType=p1  LConnTagsString=__newl0|__newl1|__newl2  RConnTagsString=__newr0|__newr1  mask(Bus){in=3, out=2, p2q=230, p3_4q=[1.0104    -0.46538], p5q=1, p6q=1}
      mask prompts: in "Number of inputs:"; out "Number of outputs:"; p2q "Voltage Rating [kV]"; p3_4q "Voltage initial guess [p.u.  rad]"; p5q "Area number"; p6q "Region number"
      mask help: Bus block.
      mask init:
      | fm_inout
      settings: AttributesFormatString="|V| =  1.0167 p.u.\\n<V  = -0.2064 rad"
      mask CallbackString: ||||fm_block|
      mask Display: plot([0 1 1 0 0],[0 0 1 1 0])
  La Arenosa 230kV : PMComponent  Tag=PSATblock  Description=Connection  PhysicalDomain=psatdomain  LeftPortType=p1  RightPortType=p1  LConnTagsString=__newl0|__newl1|__newl2|__newl3|__newl4|__newl5|__newl6|__newl7  RConnTagsString=__newr0|__newr1|__newr2|__newr3|__newr4|__newr5|__newr6|__newr7  mask(Bus){in=8, out=8, p2q=230, p3_4q=[0.98578    -0.53261], p5q=1, p6q=1}
      mask prompts: in "Number of inputs:"; out "Number of outputs:"; p2q "Voltage Rating [kV]"; p3_4q "Voltage initial guess [p.u.  rad]"; p5q "Area number"; p6q "Region number"
      mask help: Bus block.
      mask init:
      | fm_inout
      settings: AttributesFormatString="|V| =  0.9759 p.u.\\n<V  = -0.1899 rad"
      mask CallbackString: ||||fm_block|
      mask Display: plot([0 1 1 0 0],[0 0 1 1 0])
  La Arenosa 400kV : PMComponent  Tag=PSATblock  Description=Connection  PhysicalDomain=psatdomain  LeftPortType=p1  RightPortType=p1  LConnTagsString=__newl0|__newl1|__newl2|__newl3|__newl4|__newl5  RConnTagsString=__newr0|__newr1  mask(Bus){in=6, out=2, p2q=400, p3_4q=[0.97877     -0.4492], p5q=1, p6q=1}
      mask prompts: in "Number of inputs:"; out "Number of outputs:"; p2q "Voltage Rating [kV]"; p3_4q "Voltage initial guess [p.u.  rad]"; p5q "Area number"; p6q "Region number"
      mask help: Bus block.
      mask init:
      | fm_inout
      settings: AttributesFormatString="|V| =  0.9690 p.u.\\n<V  = -0.1420 rad"
      mask CallbackString: ||||fm_block|
      mask Display: plot([0 1 1 0 0],[0 0 1 1 0])
  La Arenosa 765kV : PMComponent  Tag=PSATblock  Description=Connection  PhysicalDomain=psatdomain  LeftPortType=p1  RightPortType=p1  LConnTagsString=__newl0|__newl1  RConnTagsString=__newr0|__newr1|__newr2|__newr3|__newr4  mask(Bus){in=2, out=5, p2q=765, p3_4q=[0.99847    -0.42871], p5q=1, p6q=1}
      mask prompts: in "Number of inputs:"; out "Number of outputs:"; p2q "Voltage Rating [kV]"; p3_4q "Voltage initial guess [p.u.  rad]"; p5q "Area number"; p6q "Region number"
      mask help: Bus block.
      mask init:
      | fm_inout
      settings: AttributesFormatString="|V| =  0.9725 p.u.\\n<V  = -0.1437 rad"
      mask CallbackString: ||||fm_block|
      mask Display: plot([0 1 1 0 0],[0 0 1 1 0])
  La Canoa 400kV : PMComponent  Tag=PSATblock  Description=Connection  PhysicalDomain=psatdomain  LeftPortType=p1  RightPortType=p1  LConnTagsString=__newl0|__newl1  RConnTagsString=__newr0  mask(Bus){in=2, out=1, p2q=400, p3_4q=[1.0615    -0.13875], p5q=1, p6q=1}
      mask prompts: in "Number of inputs:"; out "Number of outputs:"; p2q "Voltage Rating [kV]"; p3_4q "Voltage initial guess [p.u.  rad]"; p5q "Area number"; p6q "Region number"
      mask help: Bus block.
      mask init:
      | fm_inout
      settings: AttributesFormatString="|V| =  1.0343 p.u.\\n<V  = -0.0133 rad"
      mask CallbackString: ||||fm_block|
      mask Display: plot([0 1 1 0 0],[0 0 1 1 0])
  La Concordia : PMComponent  Tag=PSATblock  Description=Connection  PhysicalDomain=psatdomain  LeftPortType=p1  RightPortType=p1  LConnTagsString=__newl0  RConnTagsString=__newr0|__newr1  mask(Bus){in=1, out=2, p2q=115, p3_4q=[1.0023    -0.25717], p5q=1, p6q=1}
      mask prompts: in "Number of inputs:"; out "Number of outputs:"; p2q "Voltage Rating [kV]"; p3_4q "Voltage initial guess [p.u.  rad]"; p5q "Area number"; p6q "Region number"
      mask help: Bus block.
      mask init:
      | fm_inout
      settings: AttributesFormatString="|V| =  1.0138 p.u.\\n<V  =  0.4586 rad"
      mask CallbackString: ||||fm_block|
      mask Display: plot([0 1 1 0 0],[0 0 1 1 0])
  La Fria II : PMComponent  Tag=PSATblock  Description=Connection  PhysicalDomain=psatdomain  LeftPortType=p1  RightPortType=p1  LConnTagsString=__newl0  RConnTagsString=__newr0|__newr1|__newr2|__newr3  mask(Bus){in=1, out=4, p2q=115, p3_4q=[0.98444    -0.26004], p5q=1, p6q=1}
      mask prompts: in "Number of inputs:"; out "Number of outputs:"; p2q "Voltage Rating [kV]"; p3_4q "Voltage initial guess [p.u.  rad]"; p5q "Area number"; p6q "Region number"
      mask help: Bus block.
      mask init:
      | fm_inout
      settings: AttributesFormatString="|V| =  1.0176 p.u.\\n<V  =  0.4726 rad"
      mask CallbackString: ||||fm_block|
      mask Display: plot([0 1 1 0 0],[0 0 1 1 0])
  La Grita : PMComponent  Tag=PSATblock  Description=Connection  PhysicalDomain=psatdomain  LeftPortType=p1  RightPortType=p1  LConnTagsString=__newl0|__newl1|__newl2|__newl3  RConnTagsString=__newr0|__newr1|__newr2  mask(Bus){in=4, out=3, p2q=115, p3_4q=[0.98444    -0.26004], p5q=1, p6q=1}
      mask prompts: in "Number of inputs:"; out "Number of outputs:"; p2q "Voltage Rating [kV]"; p3_4q "Voltage initial guess [p.u.  rad]"; p5q "Area number"; p6q "Region number"
      mask help: Bus block.
      mask init:
      | fm_inout
      settings: AttributesFormatString="|V| =  1.0108 p.u.\\n<V  =  0.4489 rad"
      mask CallbackString: ||||fm_block|
      mask Display: plot([0 1 1 0 0],[0 0 1 1 0])
  La Horqueta 230kV : PMComponent  Tag=PSATblock  Description=Connection  PhysicalDomain=psatdomain  LeftPortType=p1  RightPortType=p1  LConnTagsString=__newl0|__newl1|__newl2|__newl3|__newl4|__newl5|__newl6|__newl7  RConnTagsString=__newr0|__newr1|__newr2|__newr3|__newr4  mask(Bus){in=8, out=5, p2q=230, p3_4q=[0.98199    -0.50182], p5q=1, p6q=1}
      mask prompts: in "Number of inputs:"; out "Number of outputs:"; p2q "Voltage Rating [kV]"; p3_4q "Voltage initial guess [p.u.  rad]"; p5q "Area number"; p6q "Region number"
      mask help: Bus block.
      mask init:
      | fm_inout
      settings: AttributesFormatString="|V| =  1.0027 p.u.\\n<V  = -0.1953 rad"
      mask CallbackString: ||||fm_block|
      mask Display: plot([0 1 1 0 0],[0 0 1 1 0])
  La Horqueta 400kV : PMComponent  Tag=PSATblock  Description=Connection  PhysicalDomain=psatdomain  LeftPortType=p1  RightPortType=p1  LConnTagsString=__newl0|__newl1|__newl2|__newl3  RConnTagsString=__newr0|__newr1  mask(Bus){in=4, out=2, p2q=400, p3_4q=[1.002    -0.44264], p5q=1, p6q=1}
      mask prompts: in "Number of inputs:"; out "Number of outputs:"; p2q "Voltage Rating [kV]"; p3_4q "Voltage initial guess [p.u.  rad]"; p5q "Area number"; p6q "Region number"
      mask help: Bus block.
      mask init:
      | fm_inout
      settings: AttributesFormatString="|V| =  1.0015 p.u.\\n<V  = -0.1547 rad"
      mask CallbackString: ||||fm_block|
      mask Display: plot([0 1 1 0 0],[0 0 1 1 0])
  La Horqueta 765kV : PMComponent  Tag=PSATblock  Description=Connection  PhysicalDomain=psatdomain  LeftPortType=p1  RightPortType=p1  LConnTagsString=__newl0|__newl1  RConnTagsString=__newr0|__newr1|__newr2|__newr3  mask(Bus){in=2, out=4, p2q=765, p3_4q=[1.05    -0.39644], p5q=1, p6q=1}
      mask prompts: in "Number of inputs:"; out "Number of outputs:"; p2q "Voltage Rating [kV]"; p3_4q "Voltage initial guess [p.u.  rad]"; p5q "Area number"; p6q "Region number"
      mask help: Bus block.
      mask init:
      | fm_inout
      settings: AttributesFormatString="|V| =  1.04   p.u.\\n<V  = -0.1439 rad"
      mask CallbackString: ||||fm_block|
      mask Display: plot([0 1 1 0 0],[0 0 1 1 0])
  La Libertad : PMComponent  Tag=PSATblock  Description=Connection  PhysicalDomain=psatdomain  LeftPortType=p1  RightPortType=p1  LConnTagsString=__newl0  RConnTagsString=__newr0|__newr1  mask(Bus){in=1, out=2, p2q=115, p3_4q=[1.0023    -0.25717], p5q=1, p6q=1}
      mask prompts: in "Number of inputs:"; out "Number of outputs:"; p2q "Voltage Rating [kV]"; p3_4q "Voltage initial guess [p.u.  rad]"; p5q "Area number"; p6q "Region number"
      mask help: Bus block.
      mask init:
      | fm_inout
      settings: AttributesFormatString="|V| =  1.0314 p.u.\\n<V  =  0.0987 rad"
      mask CallbackString: ||||fm_block|
      mask Display: plot([0 1 1 0 0],[0 0 1 1 0])
  La Pedrera : PMComponent  Tag=PSATblock  Description=Connection  PhysicalDomain=psatdomain  LeftPortType=p1  RightPortType=p1  LConnTagsString=__newl0  RConnTagsString=__newr0|__newr1  mask(Bus){in=1, out=2, p2q=115, p3_4q=[1.0023    -0.25717], p5q=1, p6q=1}
      mask prompts: in "Number of inputs:"; out "Number of outputs:"; p2q "Voltage Rating [kV]"; p3_4q "Voltage initial guess [p.u.  rad]"; p5q "Area number"; p6q "Region number"
      mask help: Bus block.
      mask init:
      | fm_inout
      settings: AttributesFormatString="|V| =  0.9948 p.u.\\n<V  =  0.4943 rad"
      mask CallbackString: ||||fm_block|
      mask Display: plot([0 1 1 0 0],[0 0 1 1 0])
  Las Claritas 230kV : PMComponent  Tag=PSATblock  Description=Connection  PhysicalDomain=psatdomain  LeftPortType=p1  RightPortType=p1  LConnTagsString=__newl0  RConnTagsString=__newr0  mask(Bus){in=1, out=1, p2q=230, p3_4q=[1.0094    -0.18727], p5q=1, p6q=1}
      mask prompts: in "Number of inputs:"; out "Number of outputs:"; p2q "Voltage Rating [kV]"; p3_4q "Voltage initial guess [p.u.  rad]"; p5q "Area number"; p6q "Region number"
      mask help: Bus block.
      mask init:
      | fm_inout
      settings: AttributesFormatString="|V| =  1.001  p.u.\\n<V  = -0.1546 rad"
      mask CallbackString: ||||fm_block|
      mask Display: plot([0 1 1 0 0],[0 0 1 1 0])
  Las Claritas 400kV : PMComponent  Tag=PSATblock  Description=Connection  PhysicalDomain=psatdomain  LeftPortType=p1  RightPortType=p1  LConnTagsString=__newl0|__newl1  RConnTagsString=__newr0  mask(Bus){in=2, out=1, p2q=400, p3_4q=[1.146    -0.14257], p5q=1, p6q=1}
      mask prompts: in "Number of inputs:"; out "Number of outputs:"; p2q "Voltage Rating [kV]"; p3_4q "Voltage initial guess [p.u.  rad]"; p5q "Area number"; p6q "Region number"
      mask help: Bus block.
      mask init:
      | fm_inout
      settings: AttributesFormatString="|V| =  1.0948 p.u.\\n<V  = -0.1112 rad"
      mask CallbackString: ||||fm_block|
      mask Display: plot([0 1 1 0 0],[0 0 1 1 0])
  Las Flores 115kV : PMComponent  Tag=PSATblock  Description=Connection  PhysicalDomain=psatdomain  LeftPortType=p1  RightPortType=p1  LConnTagsString=__newl0|__newl1  RConnTagsString=__newr0|__newr1  mask(Bus){in=2, out=2, p2q=115, p3_4q=[0.98444    -0.26004], p5q=1, p6q=1}
      mask prompts: in "Number of inputs:"; out "Number of outputs:"; p2q "Voltage Rating [kV]"; p3_4q "Voltage initial guess [p.u.  rad]"; p5q "Area number"; p6q "Region number"
      mask help: Bus block.
      mask init:
      | fm_inout
      settings: AttributesFormatString="|V| =  0.9849 p.u.\\n<V  =  0.0331 rad"
      mask CallbackString: ||||fm_block|
      mask Display: plot([0 1 1 0 0],[0 0 1 1 0])
  Las Flores 230kV : PMComponent  Tag=PSATblock  Description=Connection  PhysicalDomain=psatdomain  LeftPortType=p1  RightPortType=p1  LConnTagsString=__newl0|__newl1  RConnTagsString=__newr0  mask(Bus){in=2, out=1, p2q=230, p3_4q=[1.0163    -0.62695], p5q=1, p6q=1}
      mask prompts: in "Number of inputs:"; out "Number of outputs:"; p2q "Voltage Rating [kV]"; p3_4q "Voltage initial guess [p.u.  rad]"; p5q "Area number"; p6q "Region number"
      mask help: Bus block.
      mask init:
      | fm_inout
      settings: AttributesFormatString="|V| =  0.9955 p.u.\\n<V  =  0.0402 rad"
      mask CallbackString: ||||fm_block|
      mask Display: plot([0 1 1 0 0],[0 0 1 1 0])
  Line : PMComponent  Tag=PSATblock  Description=Power Flow  PhysicalDomain=psatdomain  LeftPortType=p1  RightPortType=p1  LConnTagsString=__newl0  RConnTagsString=__newr0  mask(Line){p3_4_5q=[100 765 60], p6q=[161], p8q=[0.012], p9q=[0.0008727], p10q=[0.013204566e-6], p13_14_15q=[25.29 22.76 25.29], p16q=on}
      mask prompts: p3_4_5q "Power, Voltage and Frequency Ratings [MVA, kV, Hz]"; p6q "Length of line [km] (0 for p.u. parameters)"; p8q "Resistance [p.u. (Ohms/km)]"; p9q "Reactance [p.u. (H/km)]"; p10q "Susceptance [p.u. (F/km)]"; p13_14_15q "Imax, Pmax and Smax [p.u., p.u., p.u.]"; p16q "Connected"
      mask help: This block defines a pi model for a tree phase line.
      mask init:
      | [xp,yp] = fm_draw('pi');
      mask CallbackString: ||||||fm_block
      mask Display:
      | plot([-1  1  1 -1 -1],[-0.2 -0.2 0.2 0.2 -0.2])
      | color('blue')
      | plot(0.35*xp,0.2*yp)
  Line1 : PMComponent  Tag=PSATblock  Description=Power Flow  PhysicalDomain=psatdomain  LeftPortType=p1  RightPortType=p1  LConnTagsString=__newl0  RConnTagsString=__newr0  mask(Line){p3_4_5q=[100 765 60], p6q=[161], p8q=[0.012], p9q=[0.0008727], p10q=[0.013204566e-6], p13_14_15q=[25.29 22.76 25.29], p16q=on}
      mask prompts: p3_4_5q "Power, Voltage and Frequency Ratings [MVA, kV, Hz]"; p6q "Length of line [km] (0 for p.u. parameters)"; p8q "Resistance [p.u. (Ohms/km)]"; p9q "Reactance [p.u. (H/km)]"; p10q "Susceptance [p.u. (F/km)]"; p13_14_15q "Imax, Pmax and Smax [p.u., p.u., p.u.]"; p16q "Connected"
      mask help: This block defines a pi model for a tree phase line.
      mask init:
      | [xp,yp] = fm_draw('pi');
      mask CallbackString: ||||||fm_block
      mask Display:
      | plot([-1  1  1 -1 -1],[-0.2 -0.2 0.2 0.2 -0.2])
      | color('blue')
      | plot(0.35*xp,0.2*yp)
  Line10 : PMComponent  Tag=PSATblock  Description=Power Flow  PhysicalDomain=psatdomain  LeftPortType=p1  RightPortType=p1  LConnTagsString=__newl0  RConnTagsString=__newr0  mask(Line){p3_4_5q=[100  230  60], p6q=43.6, p8q=[0.05], p9q=[0.001294461], p10q=[0.008941863e-6], p13_14_15q=[27.3 24.9 27.3], p16q=on}
      mask prompts: p3_4_5q "Power, Voltage and Frequency Ratings [MVA, kV, Hz]"; p6q "Length of line [km] (0 for p.u. parameters)"; p8q "Resistance [p.u. (Ohms/km)]"; p9q "Reactance [p.u. (H/km)]"; p10q "Susceptance [p.u. (F/km)]"; p13_14_15q "Imax, Pmax and Smax [p.u., p.u., p.u.]"; p16q "Connected"
      mask help: This block defines a pi model for a tree phase line.
      mask init:
      | [xp,yp] = fm_draw('pi');
      mask CallbackString: ||||||fm_block
      mask Display:
      | plot([-1  1  1 -1 -1],[-0.2 -0.2 0.2 0.2 -0.2])
      | color('blue')
      | plot(0.35*xp,0.2*yp)
  Line100 : PMComponent  Tag=PSATblock  Description=Power Flow  PhysicalDomain=psatdomain  LeftPortType=p1  RightPortType=p1  LConnTagsString=__newl0  RConnTagsString=__newr0  mask(Line){p3_4_5q=[100  230  60], p6q=109, p8q=[0.05], p9q=[0.001294461], p10q=[0.008941863e-6], p13_14_15q=[10.9 9.9 10.9], p16q=on}
      mask prompts: p3_4_5q "Power, Voltage and Frequency Ratings [MVA, kV, Hz]"; p6q "Length of line [km] (0 for p.u. parameters)"; p8q "Resistance [p.u. (Ohms/km)]"; p9q "Reactance [p.u. (H/km)]"; p10q "Susceptance [p.u. (F/km)]"; p13_14_15q "Imax, Pmax and Smax [p.u., p.u., p.u.]"; p16q "Connected"
      mask help: This block defines a pi model for a tree phase line.
      mask init:
      | [xp,yp] = fm_draw('pi');
      mask CallbackString: ||||||fm_block
      mask Display:
      | plot([-1  1  1 -1 -1],[-0.2 -0.2 0.2 0.2 -0.2])
      | color('blue')
      | plot(0.35*xp,0.2*yp)
  Line101 : PMComponent  Tag=PSATblock  Description=Power Flow  PhysicalDomain=psatdomain  LeftPortType=p1  RightPortType=p1  LConnTagsString=__newl0  RConnTagsString=__newr0  mask(Line){p3_4_5q=[100  400  60], p6q=187, p8q=[0.033806452], p9q=[0.000933966], p10q=[0.012626303e-6], p13_14_15q=[26.7 24.3 26.7], p16q=on}
      mask prompts: p3_4_5q "Power, Voltage and Frequency Ratings [MVA, kV, Hz]"; p6q "Length of line [km] (0 for p.u. parameters)"; p8q "Resistance [p.u. (Ohms/km)]"; p9q "Reactance [p.u. (H/km)]"; p10q "Susceptance [p.u. (F/km)]"; p13_14_15q "Imax, Pmax and Smax [p.u., p.u., p.u.]"; p16q "Connected"
      mask help: This block defines a pi model for a tree phase line.
      mask init:
      | [xp,yp] = fm_draw('pi');
      mask CallbackString: ||||||fm_block
      mask Display:
      | plot([-1  1  1 -1 -1],[-0.2 -0.2 0.2 0.2 -0.2])
      | color('blue')
      | plot(0.35*xp,0.2*yp)
  Line102 : PMComponent  Tag=PSATblock  Description=Power Flow  PhysicalDomain=psatdomain  LeftPortType=p1  RightPortType=p1  LConnTagsString=__newl0  RConnTagsString=__newr0  mask(Line){p3_4_5q=[100  230  60], p6q=130, p8q=[0.05], p9q=[0.001294461], p10q=[0.008941863e-6], p13_14_15q=[9.2 8.3 9.2], p16q=on}
      mask prompts: p3_4_5q "Power, Voltage and Frequency Ratings [MVA, kV, Hz]"; p6q "Length of line [km] (0 for p.u. parameters)"; p8q "Resistance [p.u. (Ohms/km)]"; p9q "Reactance [p.u. (H/km)]"; p10q "Susceptance [p.u. (F/km)]"; p13_14_15q "Imax, Pmax and Smax [p.u., p.u., p.u.]"; p16q "Connected"
      mask help: This block defines a pi model for a tree phase line.
      mask init:
      | [xp,yp] = fm_draw('pi');
      mask CallbackString: ||||||fm_block
      mask Display:
      | plot([-1  1  1 -1 -1],[-0.2 -0.2 0.2 0.2 -0.2])
      | color('blue')
      | plot(0.35*xp,0.2*yp)
  Line103 : PMComponent  Tag=PSATblock  Description=Power Flow  PhysicalDomain=psatdomain  LeftPortType=p1  RightPortType=p1  LConnTagsString=__newl0  RConnTagsString=__newr0  mask(Line){p3_4_5q=[100  230  60], p6q=300, p8q=[0.05], p9q=[0.001294461], p10q=[0.008941863e-6], p13_14_15q=[4 3.6 4], p16q=on}
      mask prompts: p3_4_5q "Power, Voltage and Frequency Ratings [MVA, kV, Hz]"; p6q "Length of line [km] (0 for p.u. parameters)"; p8q "Resistance [p.u. (Ohms/km)]"; p9q "Reactance [p.u. (H/km)]"; p10q "Susceptance [p.u. (F/km)]"; p13_14_15q "Imax, Pmax and Smax [p.u., p.u., p.u.]"; p16q "Connected"
      mask help: This block defines a pi model for a tree phase line.
      mask init:
      | [xp,yp] = fm_draw('pi');
      mask CallbackString: ||||||fm_block
      mask Display:
      | plot([-1  1  1 -1 -1],[-0.2 -0.2 0.2 0.2 -0.2])
      | color('blue')
      | plot(0.35*xp,0.2*yp)
  Line104 : PMComponent  Tag=PSATblock  Description=Power Flow  PhysicalDomain=psatdomain  LeftPortType=p1  RightPortType=p1  LConnTagsString=__newl0  RConnTagsString=__newr0  mask(Line){p3_4_5q=[100  230  60], p6q=300, p8q=[0.05], p9q=[0.001294461], p10q=[0.008941863e-6], p13_14_15q=[4 3.6 4], p16q=on}
      mask prompts: p3_4_5q "Power, Voltage and Frequency Ratings [MVA, kV, Hz]"; p6q "Length of line [km] (0 for p.u. parameters)"; p8q "Resistance [p.u. (Ohms/km)]"; p9q "Reactance [p.u. (H/km)]"; p10q "Susceptance [p.u. (F/km)]"; p13_14_15q "Imax, Pmax and Smax [p.u., p.u., p.u.]"; p16q "Connected"
      mask help: This block defines a pi model for a tree phase line.
      mask init:
      | [xp,yp] = fm_draw('pi');
      mask CallbackString: ||||||fm_block
      mask Display:
      | plot([-1  1  1 -1 -1],[-0.2 -0.2 0.2 0.2 -0.2])
      | color('blue')
      | plot(0.35*xp,0.2*yp)
  Line105 : PMComponent  Tag=PSATblock  Description=Power Flow  PhysicalDomain=psatdomain  LeftPortType=p1  RightPortType=p1  LConnTagsString=__newl0  RConnTagsString=__newr0  mask(Line){p3_4_5q=[100  230  60], p6q=68, p8q=[0.05], p9q=[0.001294461], p10q=[0.008941863e-6], p13_14_15q=[17.5 15.9 17.5], p16q=on}
      mask prompts: p3_4_5q "Power, Voltage and Frequency Ratings [MVA, kV, Hz]"; p6q "Length of line [km] (0 for p.u. parameters)"; p8q "Resistance [p.u. (Ohms/km)]"; p9q "Reactance [p.u. (H/km)]"; p10q "Susceptance [p.u. (F/km)]"; p13_14_15q "Imax, Pmax and Smax [p.u., p.u., p.u.]"; p16q "Connected"
      mask help: This block defines a pi model for a tree phase line.
      mask init:
      | [xp,yp] = fm_draw('pi');
      mask CallbackString: ||||||fm_block
      mask Display:
      | plot([-1  1  1 -1 -1],[-0.2 -0.2 0.2 0.2 -0.2])
      | color('blue')
      | plot(0.35*xp,0.2*yp)
  Line106 : PMComponent  Tag=PSATblock  Description=Power Flow  PhysicalDomain=psatdomain  LeftPortType=p1  RightPortType=p1  LConnTagsString=__newl0  RConnTagsString=__newr0  mask(Line){p3_4_5q=[100  230  60], p6q=25, p8q=[0.05], p9q=[0.001294461], p10q=[0.008941863e-6], p13_14_15q=[47.7 43.4 47.7], p16q=on}
      mask prompts: p3_4_5q "Power, Voltage and Frequency Ratings [MVA, kV, Hz]"; p6q "Length of line [km] (0 for p.u. parameters)"; p8q "Resistance [p.u. (Ohms/km)]"; p9q "Reactance [p.u. (H/km)]"; p10q "Susceptance [p.u. (F/km)]"; p13_14_15q "Imax, Pmax and Smax [p.u., p.u., p.u.]"; p16q "Connected"
      mask help: This block defines a pi model for a tree phase line.
      mask init:
      | [xp,yp] = fm_draw('pi');
      mask CallbackString: ||||||fm_block
      mask Display:
      | plot([-1  1  1 -1 -1],[-0.2 -0.2 0.2 0.2 -0.2])
      | color('blue')
      | plot(0.35*xp,0.2*yp)
  Line107 : PMComponent  Tag=PSATblock  Description=Power Flow  PhysicalDomain=psatdomain  LeftPortType=p1  RightPortType=p1  LConnTagsString=__newl0  RConnTagsString=__newr0  mask(Line){p3_4_5q=[100  230  60], p6q=152, p8q=[0.05], p9q=|, p10q=[0.008941863e-6], p13_14_15q=[7.8 7.1 7.8], p16q=on}
      mask p9q=|
      | [0.001294461
      | ]
      mask prompts: p3_4_5q "Power, Voltage and Frequency Ratings [MVA, kV, Hz]"; p6q "Length of line [km] (0 for p.u. parameters)"; p8q "Resistance [p.u. (Ohms/km)]"; p9q "Reactance [p.u. (H/km)]"; p10q "Susceptance [p.u. (F/km)]"; p13_14_15q "Imax, Pmax and Smax [p.u., p.u., p.u.]"; p16q "Connected"
      mask help: This block defines a pi model for a tree phase line.
      mask init:
      | [xp,yp] = fm_draw('pi');
      mask CallbackString: ||||||fm_block
      mask Display:
      | plot([-1  1  1 -1 -1],[-0.2 -0.2 0.2 0.2 -0.2])
      | color('blue')
      | plot(0.35*xp,0.2*yp)
  Line108 : PMComponent  Tag=PSATblock  Description=Power Flow  PhysicalDomain=psatdomain  LeftPortType=p1  RightPortType=p1  LConnTagsString=__newl0  RConnTagsString=__newr0  mask(Line){p3_4_5q=[100  230  60], p6q=152, p8q=[0.05], p9q=|, p10q=[0.008941863e-6], p13_14_15q=[7.8 7.1 7.8], p16q=on}
      mask p9q=|
      | [0.001294461
      | ]
      mask prompts: p3_4_5q "Power, Voltage and Frequency Ratings [MVA, kV, Hz]"; p6q "Length of line [km] (0 for p.u. parameters)"; p8q "Resistance [p.u. (Ohms/km)]"; p9q "Reactance [p.u. (H/km)]"; p10q "Susceptance [p.u. (F/km)]"; p13_14_15q "Imax, Pmax and Smax [p.u., p.u., p.u.]"; p16q "Connected"
      mask help: This block defines a pi model for a tree phase line.
      mask init:
      | [xp,yp] = fm_draw('pi');
      mask CallbackString: ||||||fm_block
      mask Display:
      | plot([-1  1  1 -1 -1],[-0.2 -0.2 0.2 0.2 -0.2])
      | color('blue')
      | plot(0.35*xp,0.2*yp)
  Line109 : PMComponent  Tag=PSATblock  Description=Power Flow  PhysicalDomain=psatdomain  LeftPortType=p1  RightPortType=p1  LConnTagsString=__newl0  RConnTagsString=__newr0  mask(Line){p3_4_5q=[100  230  60], p6q=150, p8q=[0.05], p9q=[0.001294461], p10q=[0.008941863e-6], p13_14_15q=[7.9 7.2 7.9], p16q=on}
      mask prompts: p3_4_5q "Power, Voltage and Frequency Ratings [MVA, kV, Hz]"; p6q "Length of line [km] (0 for p.u. parameters)"; p8q "Resistance [p.u. (Ohms/km)]"; p9q "Reactance [p.u. (H/km)]"; p10q "Susceptance [p.u. (F/km)]"; p13_14_15q "Imax, Pmax and Smax [p.u., p.u., p.u.]"; p16q "Connected"
      mask help: This block defines a pi model for a tree phase line.
      mask init:
      | [xp,yp] = fm_draw('pi');
      mask CallbackString: ||||||fm_block
      mask Display:
      | plot([-1  1  1 -1 -1],[-0.2 -0.2 0.2 0.2 -0.2])
      | color('blue')
      | plot(0.35*xp,0.2*yp)
  Line11 : PMComponent  Tag=PSATblock  Description=Power Flow  PhysicalDomain=psatdomain  LeftPortType=p1  RightPortType=p1  LConnTagsString=__newl0  RConnTagsString=__newr0  mask(Line){p3_4_5q=[100  400  60], p6q=144.2, p8q=[0.033806452], p9q=[0.000933966], p10q=[0.012626303e-6], p13_14_15q=[34.7 31.5 34.7], p16q=on}
      mask prompts: p3_4_5q "Power, Voltage and Frequency Ratings [MVA, kV, Hz]"; p6q "Length of line [km] (0 for p.u. parameters)"; p8q "Resistance [p.u. (Ohms/km)]"; p9q "Reactance [p.u. (H/km)]"; p10q "Susceptance [p.u. (F/km)]"; p13_14_15q "Imax, Pmax and Smax [p.u., p.u., p.u.]"; p16q "Connected"
      mask help: This block defines a pi model for a tree phase line.
      mask init:
      | [xp,yp] = fm_draw('pi');
      mask CallbackString: ||||||fm_block
      mask Display:
      | plot([-1  1  1 -1 -1],[-0.2 -0.2 0.2 0.2 -0.2])
      | color('blue')
      | plot(0.35*xp,0.2*yp)
  Line110 : PMComponent  Tag=PSATblock  Description=Power Flow  PhysicalDomain=psatdomain  LeftPortType=p1  RightPortType=p1  LConnTagsString=__newl0  RConnTagsString=__newr0  mask(Line){p3_4_5q=[100  230  60], p6q=134, p8q=[0.05], p9q=[0.001294461], p10q=[0.008941863e-6], p13_14_15q=[8.9 8.1 8.9], p16q=on}
      mask prompts: p3_4_5q "Power, Voltage and Frequency Ratings [MVA, kV, Hz]"; p6q "Length of line [km] (0 for p.u. parameters)"; p8q "Resistance [p.u. (Ohms/km)]"; p9q "Reactance [p.u. (H/km)]"; p10q "Susceptance [p.u. (F/km)]"; p13_14_15q "Imax, Pmax and Smax [p.u., p.u., p.u.]"; p16q "Connected"
      mask help: This block defines a pi model for a tree phase line.
      mask init:
      | [xp,yp] = fm_draw('pi');
      mask CallbackString: ||||||fm_block
      mask Display:
      | plot([-1  1  1 -1 -1],[-0.2 -0.2 0.2 0.2 -0.2])
      | color('blue')
      | plot(0.35*xp,0.2*yp)
  Line111 : PMComponent  Tag=PSATblock  Description=Power Flow  PhysicalDomain=psatdomain  LeftPortType=p1  RightPortType=p1  LConnTagsString=__newl0  RConnTagsString=__newr0  mask(Line){p3_4_5q=[100  230  60], p6q=80, p8q=[0.05], p9q=[0.001294461], p10q=[0.008941863e-6], p13_14_15q=[14.9 13.6 14.9], p16q=on}
      mask prompts: p3_4_5q "Power, Voltage and Frequency Ratings [MVA, kV, Hz]"; p6q "Length of line [km] (0 for p.u. parameters)"; p8q "Resistance [p.u. (Ohms/km)]"; p9q "Reactance [p.u. (H/km)]"; p10q "Susceptance [p.u. (F/km)]"; p13_14_15q "Imax, Pmax and Smax [p.u., p.u., p.u.]"; p16q "Connected"
      mask help: This block defines a pi model for a tree phase line.
      mask init:
      | [xp,yp] = fm_draw('pi');
      mask CallbackString: ||||||fm_block
      mask Display:
      | plot([-1  1  1 -1 -1],[-0.2 -0.2 0.2 0.2 -0.2])
      | color('blue')
      | plot(0.35*xp,0.2*yp)
  Line112 : PMComponent  Tag=PSATblock  Description=Power Flow  PhysicalDomain=psatdomain  LeftPortType=p1  RightPortType=p1  LConnTagsString=__newl0  RConnTagsString=__newr0  mask(Line){p3_4_5q=[100  230  60], p6q=50, p8q=[0.05], p9q=[0.001294461], p10q=[0.008941863e-6], p13_14_15q=[23.8 21.7 23.8], p16q=on}
      mask prompts: p3_4_5q "Power, Voltage and Frequency Ratings [MVA, kV, Hz]"; p6q "Length of line [km] (0 for p.u. parameters)"; p8q "Resistance [p.u. (Ohms/km)]"; p9q "Reactance [p.u. (H/km)]"; p10q "Susceptance [p.u. (F/km)]"; p13_14_15q "Imax, Pmax and Smax [p.u., p.u., p.u.]"; p16q "Connected"
      mask help: This block defines a pi model for a tree phase line.
      mask init:
      | [xp,yp] = fm_draw('pi');
      mask CallbackString: ||||||fm_block
      mask Display:
      | plot([-1  1  1 -1 -1],[-0.2 -0.2 0.2 0.2 -0.2])
      | color('blue')
      | plot(0.35*xp,0.2*yp)
  Line113 : PMComponent  Tag=PSATblock  Description=Power Flow  PhysicalDomain=psatdomain  LeftPortType=p1  RightPortType=p1  LConnTagsString=__newl0  RConnTagsString=__newr0  mask(Line){p3_4_5q=[100  230  60], p6q=67, p8q=[0.05], p9q=[0.001294461], p10q=[0.008941863e-6], p13_14_15q=[17.8 16.2 17.8], p16q=on}
      mask prompts: p3_4_5q "Power, Voltage and Frequency Ratings [MVA, kV, Hz]"; p6q "Length of line [km] (0 for p.u. parameters)"; p8q "Resistance [p.u. (Ohms/km)]"; p9q "Reactance [p.u. (H/km)]"; p10q "Susceptance [p.u. (F/km)]"; p13_14_15q "Imax, Pmax and Smax [p.u., p.u., p.u.]"; p16q "Connected"
      mask help: This block defines a pi model for a tree phase line.
      mask init:
      | [xp,yp] = fm_draw('pi');
      mask CallbackString: ||||||fm_block
      mask Display:
      | plot([-1  1  1 -1 -1],[-0.2 -0.2 0.2 0.2 -0.2])
      | color('blue')
      | plot(0.35*xp,0.2*yp)
  Line114 : PMComponent  Tag=PSATblock  Description=Power Flow  PhysicalDomain=psatdomain  LeftPortType=p1  RightPortType=p1  LConnTagsString=__newl0  RConnTagsString=__newr0  mask(Line){p3_4_5q=[100  230  60], p6q=44, p8q=[0.05], p9q=[0.001294461], p10q=[0.008941863e-6], p13_14_15q=[27.1 24.6 27.1], p16q=on}
      mask prompts: p3_4_5q "Power, Voltage and Frequency Ratings [MVA, kV, Hz]"; p6q "Length of line [km] (0 for p.u. parameters)"; p8q "Resistance [p.u. (Ohms/km)]"; p9q "Reactance [p.u. (H/km)]"; p10q "Susceptance [p.u. (F/km)]"; p13_14_15q "Imax, Pmax and Smax [p.u., p.u., p.u.]"; p16q "Connected"
      mask help: This block defines a pi model for a tree phase line.
      mask init:
      | [xp,yp] = fm_draw('pi');
      mask CallbackString: ||||||fm_block
      mask Display:
      | plot([-1  1  1 -1 -1],[-0.2 -0.2 0.2 0.2 -0.2])
      | color('blue')
      | plot(0.35*xp,0.2*yp)
  Line115 : PMComponent  Tag=PSATblock  Description=Power Flow  PhysicalDomain=psatdomain  LeftPortType=p1  RightPortType=p1  LConnTagsString=__newl0  RConnTagsString=__newr0  mask(Line){p3_4_5q=[100  230  60], p6q=80, p8q=[0.05], p9q=[0.001294461], p10q=[0.008941863e-6], p13_14_15q=[14.9 13.6 14.9], p16q=on}
      mask prompts: p3_4_5q "Power, Voltage and Frequency Ratings [MVA, kV, Hz]"; p6q "Length of line [km] (0 for p.u. parameters)"; p8q "Resistance [p.u. (Ohms/km)]"; p9q "Reactance [p.u. (H/km)]"; p10q "Susceptance [p.u. (F/km)]"; p13_14_15q "Imax, Pmax and Smax [p.u., p.u., p.u.]"; p16q "Connected"
      mask help: This block defines a pi model for a tree phase line.
      mask init:
      | [xp,yp] = fm_draw('pi');
      mask CallbackString: ||||||fm_block
      mask Display:
      | plot([-1  1  1 -1 -1],[-0.2 -0.2 0.2 0.2 -0.2])
      | color('blue')
      | plot(0.35*xp,0.2*yp)
  Line116 : PMComponent  Tag=PSATblock  Description=Power Flow  PhysicalDomain=psatdomain  LeftPortType=p1  RightPortType=p1  LConnTagsString=__newl0  RConnTagsString=__newr0  mask(Line){p3_4_5q=[100  230  60], p6q=13, p8q=[0.05], p9q=[0.001294461], p10q=[0.008941863e-6], p13_14_15q=[91.7 83.4 91.7], p16q=on}
      mask prompts: p3_4_5q "Power, Voltage and Frequency Ratings [MVA, kV, Hz]"; p6q "Length of line [km] (0 for p.u. parameters)"; p8q "Resistance [p.u. (Ohms/km)]"; p9q "Reactance [p.u. (H/km)]"; p10q "Susceptance [p.u. (F/km)]"; p13_14_15q "Imax, Pmax and Smax [p.u., p.u., p.u.]"; p16q "Connected"
      mask help: This block defines a pi model for a tree phase line.
      mask init:
      | [xp,yp] = fm_draw('pi');
      mask CallbackString: ||||||fm_block
      mask Display:
      | plot([-1  1  1 -1 -1],[-0.2 -0.2 0.2 0.2 -0.2])
      | color('blue')
      | plot(0.35*xp,0.2*yp)
  Line117 : PMComponent  Tag=PSATblock  Description=Power Flow  PhysicalDomain=psatdomain  LeftPortType=p1  RightPortType=p1  LConnTagsString=__newl0  RConnTagsString=__newr0  mask(Line){p3_4_5q=[100  230  60], p6q=133, p8q=[0.05], p9q=[0.001294461], p10q=[0.008941863e-6], p13_14_15q=[9 8.2 9], p16q=on}
      mask prompts: p3_4_5q "Power, Voltage and Frequency Ratings [MVA, kV, Hz]"; p6q "Length of line [km] (0 for p.u. parameters)"; p8q "Resistance [p.u. (Ohms/km)]"; p9q "Reactance [p.u. (H/km)]"; p10q "Susceptance [p.u. (F/km)]"; p13_14_15q "Imax, Pmax and Smax [p.u., p.u., p.u.]"; p16q "Connected"
      mask help: This block defines a pi model for a tree phase line.
      mask init:
      | [xp,yp] = fm_draw('pi');
      mask CallbackString: ||||||fm_block
      mask Display:
      | plot([-1  1  1 -1 -1],[-0.2 -0.2 0.2 0.2 -0.2])
      | color('blue')
      | plot(0.35*xp,0.2*yp)
  Line118 : PMComponent  Tag=PSATblock  Description=Power Flow  PhysicalDomain=psatdomain  LeftPortType=p1  RightPortType=p1  LConnTagsString=__newl0  RConnTagsString=__newr0  mask(Line){p3_4_5q=[100  230  60], p6q=95.4, p8q=[0.05], p9q=[0.001294461], p10q=[0.008941863e-6], p13_14_15q=[12.5 11.4 12.5], p16q=on}
      mask prompts: p3_4_5q "Power, Voltage and Frequency Ratings [MVA, kV, Hz]"; p6q "Length of line [km] (0 for p.u. parameters)"; p8q "Resistance [p.u. (Ohms/km)]"; p9q "Reactance [p.u. (H/km)]"; p10q "Susceptance [p.u. (F/km)]"; p13_14_15q "Imax, Pmax and Smax [p.u., p.u., p.u.]"; p16q "Connected"
      mask help: This block defines a pi model for a tree phase line.
      mask init:
      | [xp,yp] = fm_draw('pi');
      mask CallbackString: ||||||fm_block
      mask Display:
      | plot([-1  1  1 -1 -1],[-0.2 -0.2 0.2 0.2 -0.2])
      | color('blue')
      | plot(0.35*xp,0.2*yp)
  Line119 : PMComponent  Tag=PSATblock  Description=Power Flow  PhysicalDomain=psatdomain  LeftPortType=p1  RightPortType=p1  LConnTagsString=__newl0  RConnTagsString=__newr0  mask(Line){p3_4_5q=[532  230  60], p6q=224, p8q=[0.05], p9q=[0.001294461], p10q=[0.008941863e-6], p13_14_15q=[5.3 4.8 5.3], p16q=on}
      mask prompts: p3_4_5q "Power, Voltage and Frequency Ratings [MVA, kV, Hz]"; p6q "Length of line [km] (0 for p.u. parameters)"; p8q "Resistance [p.u. (Ohms/km)]"; p9q "Reactance [p.u. (H/km)]"; p10q "Susceptance [p.u. (F/km)]"; p13_14_15q "Imax, Pmax and Smax [p.u., p.u., p.u.]"; p16q "Connected"
      mask help: This block defines a pi model for a tree phase line.
      mask init:
      | [xp,yp] = fm_draw('pi');
      mask CallbackString: ||||||fm_block
      mask Display:
      | plot([-1  1  1 -1 -1],[-0.2 -0.2 0.2 0.2 -0.2])
      | color('blue')
      | plot(0.35*xp,0.2*yp)
  Line12 : PMComponent  Tag=PSATblock  Description=Power Flow  PhysicalDomain=psatdomain  LeftPortType=p1  RightPortType=p1  LConnTagsString=__newl0  RConnTagsString=__newr0  mask(Line){p3_4_5q=[100  400  60], p6q=153.9, p8q=[0.033806452], p9q=[0.000933966], p10q=[0.012626303e-6], p13_14_15q=[32.5 29.5 32.5], p16q=on}
      mask prompts: p3_4_5q "Power, Voltage and Frequency Ratings [MVA, kV, Hz]"; p6q "Length of line [km] (0 for p.u. parameters)"; p8q "Resistance [p.u. (Ohms/km)]"; p9q "Reactance [p.u. (H/km)]"; p10q "Susceptance [p.u. (F/km)]"; p13_14_15q "Imax, Pmax and Smax [p.u., p.u., p.u.]"; p16q "Connected"
      mask help: This block defines a pi model for a tree phase line.
      mask init:
      | [xp,yp] = fm_draw('pi');
      mask CallbackString: ||||||fm_block
      mask Display:
      | plot([-1  1  1 -1 -1],[-0.2 -0.2 0.2 0.2 -0.2])
      | color('blue')
      | plot(0.35*xp,0.2*yp)
  Line120 : PMComponent  Tag=PSATblock  Description=Power Flow  PhysicalDomain=psatdomain  LeftPortType=p1  RightPortType=p1  LConnTagsString=__newl0  RConnTagsString=__newr0  mask(Line){p3_4_5q=[100  230  60], p6q=80, p8q=[0.05], p9q=[0.001294461], p10q=[0.008941863e-6], p13_14_15q=[14.9 13.6 14.9], p16q=on}
      mask prompts: p3_4_5q "Power, Voltage and Frequency Ratings [MVA, kV, Hz]"; p6q "Length of line [km] (0 for p.u. parameters)"; p8q "Resistance [p.u. (Ohms/km)]"; p9q "Reactance [p.u. (H/km)]"; p10q "Susceptance [p.u. (F/km)]"; p13_14_15q "Imax, Pmax and Smax [p.u., p.u., p.u.]"; p16q "Connected"
      mask help: This block defines a pi model for a tree phase line.
      mask init:
      | [xp,yp] = fm_draw('pi');
      mask CallbackString: ||||||fm_block
      mask Display:
      | plot([-1  1  1 -1 -1],[-0.2 -0.2 0.2 0.2 -0.2])
      | color('blue')
      | plot(0.35*xp,0.2*yp)
  Line121 : PMComponent  Tag=PSATblock  Description=Power Flow  PhysicalDomain=psatdomain  LeftPortType=p1  RightPortType=p1  LConnTagsString=__newl0  RConnTagsString=__newr0  mask(Line){p3_4_5q=[532  230  60], p6q=224, p8q=[0.05], p9q=[0.001294461], p10q=[0.008941863e-6], p13_14_15q=[5.3 4.8 5.3], p16q=on}
      mask prompts: p3_4_5q "Power, Voltage and Frequency Ratings [MVA, kV, Hz]"; p6q "Length of line [km] (0 for p.u. parameters)"; p8q "Resistance [p.u. (Ohms/km)]"; p9q "Reactance [p.u. (H/km)]"; p10q "Susceptance [p.u. (F/km)]"; p13_14_15q "Imax, Pmax and Smax [p.u., p.u., p.u.]"; p16q "Connected"
      mask help: This block defines a pi model for a tree phase line.
      mask init:
      | [xp,yp] = fm_draw('pi');
      mask CallbackString: ||||||fm_block
      mask Display:
      | plot([-1  1  1 -1 -1],[-0.2 -0.2 0.2 0.2 -0.2])
      | color('blue')
      | plot(0.35*xp,0.2*yp)
  Line122 : PMComponent  Tag=PSATblock  Description=Power Flow  PhysicalDomain=psatdomain  LeftPortType=p1  RightPortType=p1  LConnTagsString=__newl0  RConnTagsString=__newr0  mask(Line){p3_4_5q=[100  230  60], p6q=80, p8q=[0.05], p9q=[0.001294461], p10q=[0.008941863e-6], p13_14_15q=[14.9 13.6 14.9], p16q=on}
      mask prompts: p3_4_5q "Power, Voltage and Frequency Ratings [MVA, kV, Hz]"; p6q "Length of line [km] (0 for p.u. parameters)"; p8q "Resistance [p.u. (Ohms/km)]"; p9q "Reactance [p.u. (H/km)]"; p10q "Susceptance [p.u. (F/km)]"; p13_14_15q "Imax, Pmax and Smax [p.u., p.u., p.u.]"; p16q "Connected"
      mask help: This block defines a pi model for a tree phase line.
      mask init:
      | [xp,yp] = fm_draw('pi');
      mask CallbackString: ||||||fm_block
      mask Display:
      | plot([-1  1  1 -1 -1],[-0.2 -0.2 0.2 0.2 -0.2])
      | color('blue')
      | plot(0.35*xp,0.2*yp)
  Line123 : PMComponent  Tag=PSATblock  Description=Power Flow  PhysicalDomain=psatdomain  LeftPortType=p1  RightPortType=p1  LConnTagsString=__newl0  RConnTagsString=__newr0  mask(Line){p3_4_5q=[100  400  60], p6q=38, p8q=[0.033806452], p9q=[0.000933966], p10q=[0.012626303e-6], p13_14_15q=[131.5 119.6 131.5], p16q=on}
      mask prompts: p3_4_5q "Power, Voltage and Frequency Ratings [MVA, kV, Hz]"; p6q "Length of line [km] (0 for p.u. parameters)"; p8q "Resistance [p.u. (Ohms/km)]"; p9q "Reactance [p.u. (H/km)]"; p10q "Susceptance [p.u. (F/km)]"; p13_14_15q "Imax, Pmax and Smax [p.u., p.u., p.u.]"; p16q "Connected"
      mask help: This block defines a pi model for a tree phase line.
      mask init:
      | [xp,yp] = fm_draw('pi');
      mask CallbackString: ||||||fm_block
      mask Display:
      | plot([-1  1  1 -1 -1],[-0.2 -0.2 0.2 0.2 -0.2])
      | color('blue')
      | plot(0.35*xp,0.2*yp)
  Line124 : PMComponent  Tag=PSATblock  Description=Power Flow  PhysicalDomain=psatdomain  LeftPortType=p1  RightPortType=p1  LConnTagsString=__newl0  RConnTagsString=__newr0  mask(Line){p3_4_5q=[100  138  60], p6q=6.2, p8q=[0.125], p9q=[0.000994719], p10q=[0.007460394e-6], p13_14_15q=[90.1 81.9 90.1], p16q=on}
      mask prompts: p3_4_5q "Power, Voltage and Frequency Ratings [MVA, kV, Hz]"; p6q "Length of line [km] (0 for p.u. parameters)"; p8q "Resistance [p.u. (Ohms/km)]"; p9q "Reactance [p.u. (H/km)]"; p10q "Susceptance [p.u. (F/km)]"; p13_14_15q "Imax, Pmax and Smax [p.u., p.u., p.u.]"; p16q "Connected"
      mask help: This block defines a pi model for a tree phase line.
      mask init:
      | [xp,yp] = fm_draw('pi');
      mask CallbackString: ||||||fm_block
      mask Display:
      | plot([-1  1  1 -1 -1],[-0.2 -0.2 0.2 0.2 -0.2])
      | color('blue')
      | plot(0.35*xp,0.2*yp)
  Line125 : PMComponent  Tag=PSATblock  Description=Power Flow  PhysicalDomain=psatdomain  LeftPortType=p1  RightPortType=p1  LConnTagsString=__newl0  RConnTagsString=__newr0  mask(Line){p3_4_5q=[100  230  60], p6q=9.8, p8q=[0.05], p9q=[0.001294461], p10q=[0.008941863e-6], p13_14_15q=[121.7 110.6 121.7], p16q=on}
      mask prompts: p3_4_5q "Power, Voltage and Frequency Ratings [MVA, kV, Hz]"; p6q "Length of line [km] (0 for p.u. parameters)"; p8q "Resistance [p.u. (Ohms/km)]"; p9q "Reactance [p.u. (H/km)]"; p10q "Susceptance [p.u. (F/km)]"; p13_14_15q "Imax, Pmax and Smax [p.u., p.u., p.u.]"; p16q "Connected"
      mask help: This block defines a pi model for a tree phase line.
      mask init:
      | [xp,yp] = fm_draw('pi');
      mask CallbackString: ||||||fm_block
      mask Display:
      | plot([-1  1  1 -1 -1],[-0.2 -0.2 0.2 0.2 -0.2])
      | color('blue')
      | plot(0.35*xp,0.2*yp)
  Line126 : PMComponent  Tag=PSATblock  Description=Power Flow  PhysicalDomain=psatdomain  LeftPortType=p1  RightPortType=p1  LConnTagsString=__newl0  RConnTagsString=__newr0  mask(Line){p3_4_5q=[100  230  60], p6q=6, p8q=[0.05], p9q=[0.001294461], p10q=[0.008941863e-6], p13_14_15q=[198.7 180.7 198.7], p16q=on}
      mask prompts: p3_4_5q "Power, Voltage and Frequency Ratings [MVA, kV, Hz]"; p6q "Length of line [km] (0 for p.u. parameters)"; p8q "Resistance [p.u. (Ohms/km)]"; p9q "Reactance [p.u. (H/km)]"; p10q "Susceptance [p.u. (F/km)]"; p13_14_15q "Imax, Pmax and Smax [p.u., p.u., p.u.]"; p16q "Connected"
      mask help: This block defines a pi model for a tree phase line.
      mask init:
      | [xp,yp] = fm_draw('pi');
      mask CallbackString: ||||||fm_block
      mask Display:
      | plot([-1  1  1 -1 -1],[-0.2 -0.2 0.2 0.2 -0.2])
      | color('blue')
      | plot(0.35*xp,0.2*yp)
  Line127 : PMComponent  Tag=PSATblock  Description=Power Flow  PhysicalDomain=psatdomain  LeftPortType=p1  RightPortType=p1  LConnTagsString=__newl0  RConnTagsString=__newr0  mask(Line){p3_4_5q=[100  230  60], p6q=16.1, p8q=[0.05], p9q=[0.001294461], p10q=[0.008941863e-6], p13_14_15q=[74.1 67.3 74.1], p16q=on}
      mask prompts: p3_4_5q "Power, Voltage and Frequency Ratings [MVA, kV, Hz]"; p6q "Length of line [km] (0 for p.u. parameters)"; p8q "Resistance [p.u. (Ohms/km)]"; p9q "Reactance [p.u. (H/km)]"; p10q "Susceptance [p.u. (F/km)]"; p13_14_15q "Imax, Pmax and Smax [p.u., p.u., p.u.]"; p16q "Connected"
      mask help: This block defines a pi model for a tree phase line.
      mask init:
      | [xp,yp] = fm_draw('pi');
      mask CallbackString: ||||||fm_block
      mask Display:
      | plot([-1  1  1 -1 -1],[-0.2 -0.2 0.2 0.2 -0.2])
      | color('blue')
      | plot(0.35*xp,0.2*yp)
  Line128 : PMComponent  Tag=PSATblock  Description=Power Flow  PhysicalDomain=psatdomain  LeftPortType=p1  RightPortType=p1  LConnTagsString=__newl0  RConnTagsString=__newr0  mask(Line){p3_4_5q=[100  138  60], p6q=6.2, p8q=[0.125], p9q=[0.000994719], p10q=[0.007460394e-6], p13_14_15q=[90.1 81.9 90.1], p16q=on}
      mask prompts: p3_4_5q "Power, Voltage and Frequency Ratings [MVA, kV, Hz]"; p6q "Length of line [km] (0 for p.u. parameters)"; p8q "Resistance [p.u. (Ohms/km)]"; p9q "Reactance [p.u. (H/km)]"; p10q "Susceptance [p.u. (F/km)]"; p13_14_15q "Imax, Pmax and Smax [p.u., p.u., p.u.]"; p16q "Connected"
      mask help: This block defines a pi model for a tree phase line.
      mask init:
      | [xp,yp] = fm_draw('pi');
      mask CallbackString: ||||||fm_block
      mask Display:
      | plot([-1  1  1 -1 -1],[-0.2 -0.2 0.2 0.2 -0.2])
      | color('blue')
      | plot(0.35*xp,0.2*yp)
  Line129 : PMComponent  Tag=PSATblock  Description=Power Flow  PhysicalDomain=psatdomain  LeftPortType=p1  RightPortType=p1  LConnTagsString=__newl0  RConnTagsString=__newr0  mask(Line){p3_4_5q=[100  230  60], p6q=9, p8q=[0.19253], p9q=[0.00021157], p10q=[0.416e-6], p13_14_15q=[810.6 736.9 810.6], p16q=on}
      mask prompts: p3_4_5q "Power, Voltage and Frequency Ratings [MVA, kV, Hz]"; p6q "Length of line [km] (0 for p.u. parameters)"; p8q "Resistance [p.u. (Ohms/km)]"; p9q "Reactance [p.u. (H/km)]"; p10q "Susceptance [p.u. (F/km)]"; p13_14_15q "Imax, Pmax and Smax [p.u., p.u., p.u.]"; p16q "Connected"
      mask help: This block defines a pi model for a tree phase cable.
      mask init:
      | [x,y] = fm_draw('circle');
      | [x1,y1] = fm_draw('semicircle');
      mask CallbackString: ||||||fm_block
      mask Display:
      | color('yellow')
      | plot(10+0.433*x,0.5+0.433*y)
      | plot(9.567+0.433*x,-0.25+0.433*y)
      | plot(10.433+0.433*x,-0.25+0.433*y)
      | color('black')
      | plot(-x1,y1)
      | plot(10+x,y,[0 10],[1 1],[0 10],[-1 -1])
  Line13 : PMComponent  Tag=PSATblock  Description=Power Flow  PhysicalDomain=psatdomain  LeftPortType=p1  RightPortType=p1  LConnTagsString=__newl0  RConnTagsString=__newr0  mask(Line){p3_4_5q=[100  400  60], p6q=169, p8q=[0.033806452], p9q=[0.000933966], p10q=[0.012626303e-6], p13_14_15q=[29.6 26.9 29.6], p16q=on}
      mask prompts: p3_4_5q "Power, Voltage and Frequency Ratings [MVA, kV, Hz]"; p6q "Length of line [km] (0 for p.u. parameters)"; p8q "Resistance [p.u. (Ohms/km)]"; p9q "Reactance [p.u. (H/km)]"; p10q "Susceptance [p.u. (F/km)]"; p13_14_15q "Imax, Pmax and Smax [p.u., p.u., p.u.]"; p16q "Connected"
      mask help: This block defines a pi model for a tree phase line.
      mask init:
      | [xp,yp] = fm_draw('pi');
      mask CallbackString: ||||||fm_block
      mask Display:
      | plot([-1  1  1 -1 -1],[-0.2 -0.2 0.2 0.2 -0.2])
      | color('blue')
      | plot(0.35*xp,0.2*yp)
  Line130 : PMComponent  Tag=PSATblock  Description=Power Flow  PhysicalDomain=psatdomain  LeftPortType=p1  RightPortType=p1  LConnTagsString=__newl0  RConnTagsString=__newr0  mask(Line){p3_4_5q=[100  138  60], p6q=4.3, p8q=[0.125], p9q=[0.000994719], p10q=[0.007460394e-6], p13_14_15q=[129.9 118.1 129.9], p16q=on}
      mask prompts: p3_4_5q "Power, Voltage and Frequency Ratings [MVA, kV, Hz]"; p6q "Length of line [km] (0 for p.u. parameters)"; p8q "Resistance [p.u. (Ohms/km)]"; p9q "Reactance [p.u. (H/km)]"; p10q "Susceptance [p.u. (F/km)]"; p13_14_15q "Imax, Pmax and Smax [p.u., p.u., p.u.]"; p16q "Connected"
      mask help: This block defines a pi model for a tree phase line.
      mask init:
      | [xp,yp] = fm_draw('pi');
      mask CallbackString: ||||||fm_block
      mask Display:
      | plot([-1  1  1 -1 -1],[-0.2 -0.2 0.2 0.2 -0.2])
      | color('blue')
      | plot(0.35*xp,0.2*yp)
  Line131 : PMComponent  Tag=PSATblock  Description=Power Flow  PhysicalDomain=psatdomain  LeftPortType=p1  RightPortType=p1  LConnTagsString=__newl0  RConnTagsString=__newr0  mask(Line){p3_4_5q=[100  230  60], p6q=12, p8q=[0.05], p9q=[0.001294461], p10q=[0.008941863e-6], p13_14_15q=[99.4 90.3 99.4], p16q=on}
      mask prompts: p3_4_5q "Power, Voltage and Frequency Ratings [MVA, kV, Hz]"; p6q "Length of line [km] (0 for p.u. parameters)"; p8q "Resistance [p.u. (Ohms/km)]"; p9q "Reactance [p.u. (H/km)]"; p10q "Susceptance [p.u. (F/km)]"; p13_14_15q "Imax, Pmax and Smax [p.u., p.u., p.u.]"; p16q "Connected"
      mask help: This block defines a pi model for a tree phase line.
      mask init:
      | [xp,yp] = fm_draw('pi');
      mask CallbackString: ||||||fm_block
      mask Display:
      | plot([-1  1  1 -1 -1],[-0.2 -0.2 0.2 0.2 -0.2])
      | color('blue')
      | plot(0.35*xp,0.2*yp)
  Line132 : PMComponent  Tag=PSATblock  Description=Power Flow  PhysicalDomain=psatdomain  LeftPortType=p1  RightPortType=p1  LConnTagsString=__newl0  RConnTagsString=__newr0  mask(Line){p3_4_5q=[100  138  60], p6q=12, p8q=[0.125], p9q=[0.000994719], p10q=[0.007460394e-6], p13_14_15q=[46.6 42.3 46.6], p16q=on}
      mask prompts: p3_4_5q "Power, Voltage and Frequency Ratings [MVA, kV, Hz]"; p6q "Length of line [km] (0 for p.u. parameters)"; p8q "Resistance [p.u. (Ohms/km)]"; p9q "Reactance [p.u. (H/km)]"; p10q "Susceptance [p.u. (F/km)]"; p13_14_15q "Imax, Pmax and Smax [p.u., p.u., p.u.]"; p16q "Connected"
      mask help: This block defines a pi model for a tree phase line.
      mask init:
      | [xp,yp] = fm_draw('pi');
      mask CallbackString: ||||||fm_block
      mask Display:
      | plot([-1  1  1 -1 -1],[-0.2 -0.2 0.2 0.2 -0.2])
      | color('blue')
      | plot(0.35*xp,0.2*yp)
